simulink model "s_c856m4k"  (R2016b)
(part 2 of 92)

      settings: AttributesFormatString=Latency = %<latency>
      mask Display:
      | port_label('input', 1, 'd');
      | port_label('output', 1, 'q');
      | disp(['Z^-', num2str(latency)]);
  pipeline20 : Subsystem  AncestorBlock=casper_library_delays/pipeline  mask(pipeline){latency=2}
      mask help:
      | An explicitly laid-out delay line to avoid mapping to SRL16s
      | for use in pipelining to help achieve timing closure.
      mask init:
      | pipeline_init(gcb,'latency',latency);
      settings: AttributesFormatString=Latency = %<latency>
      mask Display:
      | port_label('input', 1, 'd');
      | port_label('output', 1, 'q');
      | disp(['Z^-', num2str(latency)]);
  pipeline21 : Subsystem  AncestorBlock=casper_library_delays/pipeline  mask(pipeline){latency=2}
      mask help:
      | An explicitly laid-out delay line to avoid mapping to SRL16s
      | for use in pipelining to help achieve timing closure.
      mask init:
      | pipeline_init(gcb,'latency',latency);
      settings: AttributesFormatString=Latency = %<latency>
      mask Display:
      | port_label('input', 1, 'd');
      | port_label('output', 1, 'q');
      | disp(['Z^-', num2str(latency)]);
  pipeline22 : Subsystem  AncestorBlock=casper_library_delays/pipeline  mask(pipeline){latency=2}
      mask help:
      | An explicitly laid-out delay line to avoid mapping to SRL16s
      | for use in pipelining to help achieve timing closure.
      mask init:
      | pipeline_init(gcb,'latency',latency);
      settings: AttributesFormatString=Latency = %<latency>
      mask Display:
      | port_label('input', 1, 'd');
      | port_label('output', 1, 'q');
      | disp(['Z^-', num2str(latency)]);
  pipeline23 : Subsystem  AncestorBlock=casper_library_delays/pipeline  mask(pipeline){latency=2}
      mask help:
      | An explicitly laid-out delay line to avoid mapping to SRL16s
      | for use in pipelining to help achieve timing closure.
      mask init:
      | pipeline_init(gcb,'latency',latency);
      settings: AttributesFormatString=Latency = %<latency>
      mask Display:
      | port_label('input', 1, 'd');
      | port_label('output', 1, 'q');
      | disp(['Z^-', num2str(latency)]);
  pipeline24 : Subsystem  AncestorBlock=casper_library_delays/pipeline  mask(pipeline){latency=2}
      mask help:
      | An explicitly laid-out delay line to avoid mapping to SRL16s
      | for use in pipelining to help achieve timing closure.
      mask init:
      | pipeline_init(gcb,'latency',latency);
      settings: AttributesFormatString=Latency = %<latency>
      mask Display:
      | port_label('input', 1, 'd');
      | port_label('output', 1, 'q');
      | disp(['Z^-', num2str(latency)]);
  pipeline25 : Subsystem  AncestorBlock=casper_library_delays/pipeline  mask(pipeline){latency=2}
      mask help:
      | An explicitly laid-out delay line to avoid mapping to SRL16s
      | for use in pipelining to help achieve timing closure.
      mask init:
      | pipeline_init(gcb,'latency',latency);
      settings: AttributesFormatString=Latency = %<latency>
      mask Display:
      | port_label('input', 1, 'd');
      | port_label('output', 1, 'q');
      | disp(['Z^-', num2str(latency)]);
  pipeline26 : Subsystem  AncestorBlock=casper_library_delays/pipeline  mask(pipeline){latency=2}
      mask help:
      | An explicitly laid-out delay line to avoid mapping to SRL16s
      | for use in pipelining to help achieve timing closure.
      mask init:
      | pipeline_init(gcb,'latency',latency);
      settings: AttributesFormatString=Latency = %<latency>
      mask Display:
      | port_label('input', 1, 'd');
      | port_label('output', 1, 'q');
      | disp(['Z^-', num2str(latency)]);
  pipeline27 : Subsystem  AncestorBlock=casper_library_delays/pipeline  mask(pipeline){latency=2}
      mask help:
      | An explicitly laid-out delay line to avoid mapping to SRL16s
      | for use in pipelining to help achieve timing closure.
      mask init:
      | pipeline_init(gcb,'latency',latency);
      settings: AttributesFormatString=Latency = %<latency>
      mask Display:
      | port_label('input', 1, 'd');
      | port_label('output', 1, 'q');
      | disp(['Z^-', num2str(latency)]);
  pipeline28 : Subsystem  AncestorBlock=casper_library_delays/pipeline  mask(pipeline){latency=2}
      mask help:
      | An explicitly laid-out delay line to avoid mapping to SRL16s
      | for use in pipelining to help achieve timing closure.
      mask init:
      | pipeline_init(gcb,'latency',latency);
      settings: AttributesFormatString=Latency = %<latency>
      mask Display:
      | port_label('input', 1, 'd');
      | port_label('output', 1, 'q');
      | disp(['Z^-', num2str(latency)]);
  pipeline29 : Subsystem  AncestorBlock=casper_library_delays/pipeline  mask(pipeline){latency=2}
      mask help:
      | An explicitly laid-out delay line to avoid mapping to SRL16s
      | for use in pipelining to help achieve timing closure.
      mask init:
      | pipeline_init(gcb,'latency',latency);
      settings: AttributesFormatString=Latency = %<latency>
      mask Display:
      | port_label('input', 1, 'd');
      | port_label('output', 1, 'q');
      | disp(['Z^-', num2str(latency)]);
  pipeline3 : Subsystem  AncestorBlock=casper_library_delays/pipeline  mask(pipeline){latency=2}
      mask help:
      | An explicitly laid-out delay line to avoid mapping to SRL16s
      | for use in pipelining to help achieve timing closure.
      mask init:
      | pipeline_init(gcb,'latency',latency);
      settings: AttributesFormatString=Latency = %<latency>
      mask Display:
      | port_label('input', 1, 'd');
      | port_label('output', 1, 'q');
      | disp(['Z^-', num2str(latency)]);
  pipeline30 : Subsystem  AncestorBlock=casper_library_delays/pipeline  mask(pipeline){latency=2}
      mask help:
      | An explicitly laid-out delay line to avoid mapping to SRL16s
      | for use in pipelining to help achieve timing closure.
      mask init:
      | pipeline_init(gcb,'latency',latency);
      settings: AttributesFormatString=Latency = %<latency>
      mask Display:
      | port_label('input', 1, 'd');
      | port_label('output', 1, 'q');
      | disp(['Z^-', num2str(latency)]);
  pipeline31 : Subsystem  AncestorBlock=casper_library_delays/pipeline  mask(pipeline){latency=2}
      mask help:
      | An explicitly laid-out delay line to avoid mapping to SRL16s
      | for use in pipelining to help achieve timing closure.
      mask init:
      | pipeline_init(gcb,'latency',latency);
      settings: AttributesFormatString=Latency = %<latency>
      mask Display:
      | port_label('input', 1, 'd');
      | port_label('output', 1, 'q');
      | disp(['Z^-', num2str(latency)]);
  pipeline32 : Subsystem  AncestorBlock=casper_library_delays/pipeline  mask(pipeline){latency=2}
      mask help:
      | An explicitly laid-out delay line to avoid mapping to SRL16s
      | for use in pipelining to help achieve timing closure.
      mask init:
      | pipeline_init(gcb,'latency',latency);
      settings: AttributesFormatString=Latency = %<latency>
      mask Display:
      | port_label('input', 1, 'd');
      | port_label('output', 1, 'q');
      | disp(['Z^-', num2str(latency)]);
  pipeline33 : Subsystem  AncestorBlock=casper_library_delays/pipeline  mask(pipeline){latency=2}
      mask help:
      | An explicitly laid-out delay line to avoid mapping to SRL16s
      | for use in pipelining to help achieve timing closure.
      mask init:
      | pipeline_init(gcb,'latency',latency);
      settings: AttributesFormatString=Latency = %<latency>
      mask Display:
      | port_label('input', 1, 'd');
      | port_label('output', 1, 'q');
      | disp(['Z^-', num2str(latency)]);
  pipeline34 : Subsystem  AncestorBlock=casper_library_delays/pipeline  mask(pipeline){latency=2}
      mask help:
      | An explicitly laid-out delay line to avoid mapping to SRL16s
      | for use in pipelining to help achieve timing closure.
      mask init:
      | pipeline_init(gcb,'latency',latency);
      settings: AttributesFormatString=Latency = %<latency>
      mask Display:
      | port_label('input', 1, 'd');
      | port_label('output', 1, 'q');
      | disp(['Z^-', num2str(latency)]);
  pipeline35 : Subsystem  AncestorBlock=casper_library_delays/pipeline  mask(pipeline){latency=2}
      mask help:
      | An explicitly laid-out delay line to avoid mapping to SRL16s
      | for use in pipelining to help achieve timing closure.
      mask init:
      | pipeline_init(gcb,'latency',latency);
      settings: AttributesFormatString=Latency = %<latency>
      mask Display:
      | port_label('input', 1, 'd');
      | port_label('output', 1, 'q');
      | disp(['Z^-', num2str(latency)]);
  pipeline36 : Subsystem  AncestorBlock=casper_library_delays/pipeline  mask(pipeline){latency=2}
      mask help:
      | An explicitly laid-out delay line to avoid mapping to SRL16s
      | for use in pipelining to help achieve timing closure.
      mask init:
      | pipeline_init(gcb,'latency',latency);
      settings: AttributesFormatString=Latency = %<latency>
      mask Display:
      | port_label('input', 1, 'd');
      | port_label('output', 1, 'q');
      | disp(['Z^-', num2str(latency)]);
  pipeline37 : Subsystem  AncestorBlock=casper_library_delays/pipeline  mask(pipeline){latency=2}
      mask help:
      | An explicitly laid-out delay line to avoid mapping to SRL16s
      | for use in pipelining to help achieve timing closure.
      mask init:
      | pipeline_init(gcb,'latency',latency);
      settings: AttributesFormatString=Latency = %<latency>
      mask Display:
      | port_label('input', 1, 'd');
      | port_label('output', 1, 'q');
      | disp(['Z^-', num2str(latency)]);
  pipeline38 : Subsystem  AncestorBlock=casper_library_delays/pipeline  mask(pipeline){latency=2}
      mask help:
      | An explicitly laid-out delay line to avoid mapping to SRL16s
      | for use in pipelining to help achieve timing closure.
      mask init:
      | pipeline_init(gcb,'latency',latency);
      settings: AttributesFormatString=Latency = %<latency>
      mask Display:
      | port_label('input', 1, 'd');
      | port_label('output', 1, 'q');
      | disp(['Z^-', num2str(latency)]);
  pipeline39 : Subsystem  AncestorBlock=casper_library_delays/pipeline  mask(pipeline){latency=2}
      mask help:
      | An explicitly laid-out delay line to avoid mapping to SRL16s
      | for use in pipelining to help achieve timing closure.
      mask init:
      | pipeline_init(gcb,'latency',latency);
      settings: AttributesFormatString=Latency = %<latency>
      mask Display:
      | port_label('input', 1, 'd');
      | port_label('output', 1, 'q');
      | disp(['Z^-', num2str(latency)]);
  pipeline4 : Subsystem  AncestorBlock=casper_library_delays/pipeline  mask(pipeline){latency=2}
      mask help:
      | An explicitly laid-out delay line to avoid mapping to SRL16s
      | for use in pipelining to help achieve timing closure.
      mask init:
      | pipeline_init(gcb,'latency',latency);
      settings: AttributesFormatString=Latency = %<latency>
      mask Display:
      | port_label('input', 1, 'd');
      | port_label('output', 1, 'q');
      | disp(['Z^-', num2str(latency)]);
  pipeline40 : Subsystem  AncestorBlock=casper_library_delays/pipeline  mask(pipeline){latency=2}
      mask help:
      | An explicitly laid-out delay line to avoid mapping to SRL16s
      | for use in pipelining to help achieve timing closure.
      mask init:
      | pipeline_init(gcb,'latency',latency);
      settings: AttributesFormatString=Latency = %<latency>
      mask Display:
      | port_label('input', 1, 'd');
      | port_label('output', 1, 'q');
      | disp(['Z^-', num2str(latency)]);
  pipeline41 : Subsystem  AncestorBlock=casper_library_delays/pipeline  mask(pipeline){latency=2}
      mask help:
      | An explicitly laid-out delay line to avoid mapping to SRL16s
      | for use in pipelining to help achieve timing closure.
      mask init:
      | pipeline_init(gcb,'latency',latency);
      settings: AttributesFormatString=Latency = %<latency>
      mask Display:
      | port_label('input', 1, 'd');
      | port_label('output', 1, 'q');
      | disp(['Z^-', num2str(latency)]);
  pipeline42 : Subsystem  AncestorBlock=casper_library_delays/pipeline  mask(pipeline){latency=2}
      mask help:
      | An explicitly laid-out delay line to avoid mapping to SRL16s
      | for use in pipelining to help achieve timing closure.
      mask init:
      | pipeline_init(gcb,'latency',latency);
      settings: AttributesFormatString=Latency = %<latency>
      mask Display:
      | port_label('input', 1, 'd');
      | port_label('output', 1, 'q');
      | disp(['Z^-', num2str(latency)]);
  pipeline43 : Subsystem  AncestorBlock=casper_library_delays/pipeline  mask(pipeline){latency=2}
      mask help:
      | An explicitly laid-out delay line to avoid mapping to SRL16s
      | for use in pipelining to help achieve timing closure.
      mask init:
      | pipeline_init(gcb,'latency',latency);
      settings: AttributesFormatString=Latency = %<latency>
      mask Display:
      | port_label('input', 1, 'd');
      | port_label('output', 1, 'q');
      | disp(['Z^-', num2str(latency)]);
  pipeline44 : Subsystem  AncestorBlock=casper_library_delays/pipeline  mask(pipeline){latency=2}
      mask help:
      | An explicitly laid-out delay line to avoid mapping to SRL16s
      | for use in pipelining to help achieve timing closure.
      mask init:
      | pipeline_init(gcb,'latency',latency);
      settings: AttributesFormatString=Latency = %<latency>
      mask Display:
      | port_label('input', 1, 'd');
      | port_label('output', 1, 'q');
      | disp(['Z^-', num2str(latency)]);
  pipeline45 : Subsystem  AncestorBlock=casper_library_delays/pipeline  mask(pipeline){latency=2}
      mask help:
      | An explicitly laid-out delay line to avoid mapping to SRL16s
      | for use in pipelining to help achieve timing closure.
      mask init:
      | pipeline_init(gcb,'latency',latency);
      settings: AttributesFormatString=Latency = %<latency>
      mask Display:
      | port_label('input', 1, 'd');
      | port_label('output', 1, 'q');
      | disp(['Z^-', num2str(latency)]);
  pipeline46 : Subsystem  AncestorBlock=casper_library_delays/pipeline  mask(pipeline){latency=2}
      mask help:
      | An explicitly laid-out delay line to avoid mapping to SRL16s
      | for use in pipelining to help achieve timing closure.
      mask init:
      | pipeline_init(gcb,'latency',latency);
      settings: AttributesFormatString=Latency = %<latency>
      mask Display:
      | port_label('input', 1, 'd');
      | port_label('output', 1, 'q');
      | disp(['Z^-', num2str(latency)]);
  pipeline47 : Subsystem  AncestorBlock=casper_library_delays/pipeline  mask(pipeline){latency=2}
      mask help:
      | An explicitly laid-out delay line to avoid mapping to SRL16s
      | for use in pipelining to help achieve timing closure.
      mask init:
      | pipeline_init(gcb,'latency',latency);
      settings: AttributesFormatString=Latency = %<latency>
      mask Display:
      | port_label('input', 1, 'd');
      | port_label('output', 1, 'q');
      | disp(['Z^-', num2str(latency)]);
  pipeline48 : Subsystem  AncestorBlock=casper_library_delays/pipeline  mask(pipeline){latency=2}
      mask help:
      | An explicitly laid-out delay line to avoid mapping to SRL16s
      | for use in pipelining to help achieve timing closure.
      mask init:
      | pipeline_init(gcb,'latency',latency);
      settings: AttributesFormatString=Latency = %<latency>
      mask Display:
      | port_label('input', 1, 'd');
      | port_label('output', 1, 'q');
      | disp(['Z^-', num2str(latency)]);
  pipeline49 : Subsystem  AncestorBlock=casper_library_delays/pipeline  mask(pipeline){latency=2}
      mask help:
      | An explicitly laid-out delay line to avoid mapping to SRL16s
      | for use in pipelining to help achieve timing closure.
      mask init:
      | pipeline_init(gcb,'latency',latency);
      settings: AttributesFormatString=Latency = %<latency>
      mask Display:
      | port_label('input', 1, 'd');
      | port_label('output', 1, 'q');
      | disp(['Z^-', num2str(latency)]);
  pipeline5 : Subsystem  AncestorBlock=casper_library_delays/pipeline  mask(pipeline){latency=2}
      mask help:
      | An explicitly laid-out delay line to avoid mapping to SRL16s
      | for use in pipelining to help achieve timing closure.
      mask init:
      | pipeline_init(gcb,'latency',latency);
      settings: AttributesFormatString=Latency = %<latency>
      mask Display:
      | port_label('input', 1, 'd');
      | port_label('output', 1, 'q');
      | disp(['Z^-', num2str(latency)]);
  pipeline50 : Subsystem  AncestorBlock=casper_library_delays/pipeline  mask(pipeline){latency=2}
      mask help:
      | An explicitly laid-out delay line to avoid mapping to SRL16s
      | for use in pipelining to help achieve timing closure.
      mask init:
      | pipeline_init(gcb,'latency',latency);
      settings: AttributesFormatString=Latency = %<latency>
      mask Display:
      | port_label('input', 1, 'd');
      | port_label('output', 1, 'q');
      | disp(['Z^-', num2str(latency)]);
  pipeline51 : Subsystem  AncestorBlock=casper_library_delays/pipeline  mask(pipeline){latency=2}
      mask help:
      | An explicitly laid-out delay line to avoid mapping to SRL16s
      | for use in pipelining to help achieve timing closure.
      mask init:
      | pipeline_init(gcb,'latency',latency);
      settings: AttributesFormatString=Latency = %<latency>
      mask Display:
      | port_label('input', 1, 'd');
      | port_label('output', 1, 'q');
      | disp(['Z^-', num2str(latency)]);
  pipeline52 : Subsystem  AncestorBlock=casper_library_delays/pipeline  mask(pipeline){latency=2}
      mask help:
      | An explicitly laid-out delay line to avoid mapping to SRL16s
      | for use in pipelining to help achieve timing closure.
      mask init:
      | pipeline_init(gcb,'latency',latency);
      settings: AttributesFormatString=Latency = %<latency>
      mask Display:
      | port_label('input', 1, 'd');
      | port_label('output', 1, 'q');
      | disp(['Z^-', num2str(latency)]);
  pipeline53 : Subsystem  AncestorBlock=casper_library_delays/pipeline  mask(pipeline){latency=2}
      mask help:
      | An explicitly laid-out delay line to avoid mapping to SRL16s
      | for use in pipelining to help achieve timing closure.
      mask init:
      | pipeline_init(gcb,'latency',latency);
      settings: AttributesFormatString=Latency = %<latency>
      mask Display:
      | port_label('input', 1, 'd');
      | port_label('output', 1, 'q');
      | disp(['Z^-', num2str(latency)]);
  pipeline54 : Subsystem  AncestorBlock=casper_library_delays/pipeline  mask(pipeline){latency=2}
      mask help:
      | An explicitly laid-out delay line to avoid mapping to SRL16s
      | for use in pipelining to help achieve timing closure.
      mask init:
      | pipeline_init(gcb,'latency',latency);
      settings: AttributesFormatString=Latency = %<latency>
      mask Display:
      | port_label('input', 1, 'd');
      | port_label('output', 1, 'q');
      | disp(['Z^-', num2str(latency)]);
  pipeline55 : Subsystem  AncestorBlock=casper_library_delays/pipeline  mask(pipeline){latency=2}
      mask help:
      | An explicitly laid-out delay line to avoid mapping to SRL16s
      | for use in pipelining to help achieve timing closure.
      mask init:
      | pipeline_init(gcb,'latency',latency);
      settings: AttributesFormatString=Latency = %<latency>
      mask Display:
      | port_label('input', 1, 'd');
      | port_label('output', 1, 'q');
      | disp(['Z^-', num2str(latency)]);
  pipeline56 : Subsystem  AncestorBlock=casper_library_delays/pipeline  mask(pipeline){latency=2}
      mask help:
      | An explicitly laid-out delay line to avoid mapping to SRL16s
      | for use in pipelining to help achieve timing closure.
      mask init:
      | pipeline_init(gcb,'latency',latency);
      settings: AttributesFormatString=Latency = %<latency>
      mask Display:
      | port_label('input', 1, 'd');
      | port_label('output', 1, 'q');
      | disp(['Z^-', num2str(latency)]);
  pipeline57 : Subsystem  AncestorBlock=casper_library_delays/pipeline  mask(pipeline){latency=2}
      mask help:
      | An explicitly laid-out delay line to avoid mapping to SRL16s
      | for use in pipelining to help achieve timing closure.
      mask init:
      | pipeline_init(gcb,'latency',latency);
      settings: AttributesFormatString=Latency = %<latency>
      mask Display:
      | port_label('input', 1, 'd');
      | port_label('output', 1, 'q');
      | disp(['Z^-', num2str(latency)]);
  pipeline58 : Subsystem  AncestorBlock=casper_library_delays/pipeline  mask(pipeline){latency=2}
      mask help:
      | An explicitly laid-out delay line to avoid mapping to SRL16s
      | for use in pipelining to help achieve timing closure.
      mask init:
      | pipeline_init(gcb,'latency',latency);
      settings: AttributesFormatString=Latency = %<latency>
      mask Display:
      | port_label('input', 1, 'd');
      | port_label('output', 1, 'q');
      | disp(['Z^-', num2str(latency)]);
  pipeline59 : Subsystem  AncestorBlock=casper_library_delays/pipeline  mask(pipeline){latency=2}
      mask help:
      | An explicitly laid-out delay line to avoid mapping to SRL16s
      | for use in pipelining to help achieve timing closure.
      mask init:
      | pipeline_init(gcb,'latency',latency);
      settings: AttributesFormatString=Latency = %<latency>
      mask Display:
      | port_label('input', 1, 'd');
      | port_label('output', 1, 'q');
      | disp(['Z^-', num2str(latency)]);
  pipeline6 : Subsystem  AncestorBlock=casper_library_delays/pipeline  mask(pipeline){latency=2}
      mask help:
      | An explicitly laid-out delay line to avoid mapping to SRL16s
      | for use in pipelining to help achieve timing closure.
      mask init:
      | pipeline_init(gcb,'latency',latency);
      settings: AttributesFormatString=Latency = %<latency>
      mask Display:
      | port_label('input', 1, 'd');
      | port_label('output', 1, 'q');
      | disp(['Z^-', num2str(latency)]);
  pipeline60 : Subsystem  AncestorBlock=casper_library_delays/pipeline  mask(pipeline){latency=2}
      mask help:
      | An explicitly laid-out delay line to avoid mapping to SRL16s
      | for use in pipelining to help achieve timing closure.
      mask init:
      | pipeline_init(gcb,'latency',latency);
      settings: AttributesFormatString=Latency = %<latency>
      mask Display:
      | port_label('input', 1, 'd');
      | port_label('output', 1, 'q');
      | disp(['Z^-', num2str(latency)]);
  pipeline61 : Subsystem  AncestorBlock=casper_library_delays/pipeline  mask(pipeline){latency=2}
      mask help:
      | An explicitly laid-out delay line to avoid mapping to SRL16s
      | for use in pipelining to help achieve timing closure.
      mask init:
      | pipeline_init(gcb,'latency',latency);
      settings: AttributesFormatString=Latency = %<latency>
      mask Display:
      | port_label('input', 1, 'd');
      | port_label('output', 1, 'q');
      | disp(['Z^-', num2str(latency)]);
  pipeline62 : Subsystem  AncestorBlock=casper_library_delays/pipeline  mask(pipeline){latency=2}
      mask help:
      | An explicitly laid-out delay line to avoid mapping to SRL16s
      | for use in pipelining to help achieve timing closure.
      mask init:
      | pipeline_init(gcb,'latency',latency);
      settings: AttributesFormatString=Latency = %<latency>
      mask Display:
      | port_label('input', 1, 'd');
      | port_label('output', 1, 'q');
      | disp(['Z^-', num2str(latency)]);
  pipeline63 : Subsystem  AncestorBlock=casper_library_delays/pipeline  mask(pipeline){latency=2}
      mask help:
      | An explicitly laid-out delay line to avoid mapping to SRL16s
      | for use in pipelining to help achieve timing closure.
      mask init:
      | pipeline_init(gcb,'latency',latency);
      settings: AttributesFormatString=Latency = %<latency>
      mask Display:
      | port_label('input', 1, 'd');
      | port_label('output', 1, 'q');
      | disp(['Z^-', num2str(latency)]);
  pipeline64 : Subsystem  AncestorBlock=casper_library_delays/pipeline  mask(pipeline){latency=2}
      mask help:
      | An explicitly laid-out delay line to avoid mapping to SRL16s
      | for use in pipelining to help achieve timing closure.
      mask init:
      | pipeline_init(gcb,'latency',latency);
      settings: AttributesFormatString=Latency = %<latency>
      mask Display:
      | port_label('input', 1, 'd');
      | port_label('output', 1, 'q');
      | disp(['Z^-', num2str(latency)]);
  pipeline65 : Subsystem  AncestorBlock=casper_library_delays/pipeline  mask(pipeline){latency=1}
      mask help:
      | An explicitly laid-out delay line to avoid mapping to SRL16s
      | for use in pipelining to help achieve timing closure.
      mask init:
      | pipeline_init(gcb,'latency',latency);
      settings: AttributesFormatString=Latency = %<latency>
      mask Display:
      | port_label('input', 1, 'd');
      | port_label('output', 1, 'q');
      | disp(['Z^-', num2str(latency)]);
  pipeline66 : Subsystem  AncestorBlock=casper_library_delays/pipeline  mask(pipeline){latency=2}
      mask help:
      | An explicitly laid-out delay line to avoid mapping to SRL16s
      | for use in pipelining to help achieve timing closure.
      mask init:
      | pipeline_init(gcb,'latency',latency);
      settings: AttributesFormatString=Latency = %<latency>
      mask Display:
      | port_label('input', 1, 'd');
      | port_label('output', 1, 'q');
      | disp(['Z^-', num2str(latency)]);
  pipeline67 : Subsystem  AncestorBlock=casper_library_delays/pipeline  mask(pipeline){latency=2}
      mask help:
      | An explicitly laid-out delay line to avoid mapping to SRL16s
      | for use in pipelining to help achieve timing closure.
      mask init:
      | pipeline_init(gcb,'latency',latency);
      settings: AttributesFormatString=Latency = %<latency>
      mask Display:
      | port_label('input', 1, 'd');
      | port_label('output', 1, 'q');
      | disp(['Z^-', num2str(latency)]);
  pipeline68 : Subsystem  AncestorBlock=casper_library_delays/pipeline  mask(pipeline){latency=2}
      mask help:
      | An explicitly laid-out delay line to avoid mapping to SRL16s
      | for use in pipelining to help achieve timing closure.
      mask init:
      | pipeline_init(gcb,'latency',latency);
      settings: AttributesFormatString=Latency = %<latency>
      mask Display:
      | port_label('input', 1, 'd');
      | port_label('output', 1, 'q');
      | disp(['Z^-', num2str(latency)]);
  pipeline69 : Subsystem  AncestorBlock=casper_library_delays/pipeline  mask(pipeline){latency=2}
      mask help:
      | An explicitly laid-out delay line to avoid mapping to SRL16s
      | for use in pipelining to help achieve timing closure.
      mask init:
      | pipeline_init(gcb,'latency',latency);
      settings: AttributesFormatString=Latency = %<latency>
      mask Display:
      | port_label('input', 1, 'd');
      | port_label('output', 1, 'q');
      | disp(['Z^-', num2str(latency)]);
  pipeline7 : Subsystem  AncestorBlock=casper_library_delays/pipeline  mask(pipeline){latency=2}
      mask help:
      | An explicitly laid-out delay line to avoid mapping to SRL16s
      | for use in pipelining to help achieve timing closure.
      mask init:
      | pipeline_init(gcb,'latency',latency);
      settings: AttributesFormatString=Latency = %<latency>
      mask Display:
      | port_label('input', 1, 'd');
      | port_label('output', 1, 'q');
      | disp(['Z^-', num2str(latency)]);
  pipeline70 : Subsystem  AncestorBlock=casper_library_delays/pipeline  mask(pipeline){latency=2}
      mask help:
      | An explicitly laid-out delay line to avoid mapping to SRL16s
      | for use in pipelining to help achieve timing closure.
      mask init:
      | pipeline_init(gcb,'latency',latency);
      settings: AttributesFormatString=Latency = %<latency>
      mask Display:
      | port_label('input', 1, 'd');
      | port_label('output', 1, 'q');
      | disp(['Z^-', num2str(latency)]);
  pipeline71 : Subsystem  AncestorBlock=casper_library_delays/pipeline  mask(pipeline){latency=2}
      mask help:
      | An explicitly laid-out delay line to avoid mapping to SRL16s
      | for use in pipelining to help achieve timing closure.
      mask init:
      | pipeline_init(gcb,'latency',latency);
      settings: AttributesFormatString=Latency = %<latency>
      mask Display:
      | port_label('input', 1, 'd');
      | port_label('output', 1, 'q');
      | disp(['Z^-', num2str(latency)]);
  pipeline72 : Subsystem  AncestorBlock=casper_library_delays/pipeline  mask(pipeline){latency=2}
      mask help:
      | An explicitly laid-out delay line to avoid mapping to SRL16s
      | for use in pipelining to help achieve timing closure.
      mask init:
      | pipeline_init(gcb,'latency',latency);
      settings: AttributesFormatString=Latency = %<latency>
      mask Display:
      | port_label('input', 1, 'd');
      | port_label('output', 1, 'q');
      | disp(['Z^-', num2str(latency)]);
  pipeline73 : Subsystem  AncestorBlock=casper_library_delays/pipeline  mask(pipeline){latency=2}
      mask help:
      | An explicitly laid-out delay line to avoid mapping to SRL16s
      | for use in pipelining to help achieve timing closure.
      mask init:
      | pipeline_init(gcb,'latency',latency);
      settings: AttributesFormatString=Latency = %<latency>
      mask Display:
      | port_label('input', 1, 'd');
      | port_label('output', 1, 'q');
      | disp(['Z^-', num2str(latency)]);
  pipeline74 : Subsystem  AncestorBlock=casper_library_delays/pipeline  mask(pipeline){latency=2}
      mask help:
      | An explicitly laid-out delay line to avoid mapping to SRL16s
      | for use in pipelining to help achieve timing closure.
      mask init:
      | pipeline_init(gcb,'latency',latency);
      settings: AttributesFormatString=Latency = %<latency>
      mask Display:
      | port_label('input', 1, 'd');
      | port_label('output', 1, 'q');
      | disp(['Z^-', num2str(latency)]);
  pipeline75 : Subsystem  AncestorBlock=casper_library_delays/pipeline  mask(pipeline){latency=2}
      mask help:
      | An explicitly laid-out delay line to avoid mapping to SRL16s
      | for use in pipelining to help achieve timing closure.
      mask init:
      | pipeline_init(gcb,'latency',latency);
      settings: AttributesFormatString=Latency = %<latency>
      mask Display:
      | port_label('input', 1, 'd');
      | port_label('output', 1, 'q');
      | disp(['Z^-', num2str(latency)]);
  pipeline76 : Subsystem  AncestorBlock=casper_library_delays/pipeline  mask(pipeline){latency=2}
      mask help:
      | An explicitly laid-out delay line to avoid mapping to SRL16s
      | for use in pipelining to help achieve timing closure.
      mask init:
      | pipeline_init(gcb,'latency',latency);
      settings: AttributesFormatString=Latency = %<latency>
      mask Display:
      | port_label('input', 1, 'd');
      | port_label('output', 1, 'q');
      | disp(['Z^-', num2str(latency)]);
  pipeline77 : Subsystem  AncestorBlock=casper_library_delays/pipeline  mask(pipeline){latency=2}
      mask help:
      | An explicitly laid-out delay line to avoid mapping to SRL16s
      | for use in pipelining to help achieve timing closure.
      mask init:
      | pipeline_init(gcb,'latency',latency);
      settings: AttributesFormatString=Latency = %<latency>
      mask Display:
      | port_label('input', 1, 'd');
      | port_label('output', 1, 'q');
      | disp(['Z^-', num2str(latency)]);
  pipeline78 : Subsystem  AncestorBlock=casper_library_delays/pipeline  mask(pipeline){latency=2}
      mask help:
      | An explicitly laid-out delay line to avoid mapping to SRL16s
      | for use in pipelining to help achieve timing closure.
      mask init:
      | pipeline_init(gcb,'latency',latency);
      settings: AttributesFormatString=Latency = %<latency>
      mask Display:
      | port_label('input', 1, 'd');
      | port_label('output', 1, 'q');
      | disp(['Z^-', num2str(latency)]);
  pipeline79 : Subsystem  AncestorBlock=casper_library_delays/pipeline  mask(pipeline){latency=2}
      mask help:
      | An explicitly laid-out delay line to avoid mapping to SRL16s
      | for use in pipelining to help achieve timing closure.
      mask init:
      | pipeline_init(gcb,'latency',latency);
      settings: AttributesFormatString=Latency = %<latency>
      mask Display:
      | port_label('input', 1, 'd');
      | port_label('output', 1, 'q');
      | disp(['Z^-', num2str(latency)]);
  pipeline8 : Subsystem  AncestorBlock=casper_library_delays/pipeline  mask(pipeline){latency=2}
      mask help:
      | An explicitly laid-out delay line to avoid mapping to SRL16s
      | for use in pipelining to help achieve timing closure.
      mask init:
      | pipeline_init(gcb,'latency',latency);
      settings: AttributesFormatString=Latency = %<latency>
      mask Display:
      | port_label('input', 1, 'd');
      | port_label('output', 1, 'q');
      | disp(['Z^-', num2str(latency)]);
  pipeline80 : Subsystem  AncestorBlock=casper_library_delays/pipeline  mask(pipeline){latency=2}
      mask help:
      | An explicitly laid-out delay line to avoid mapping to SRL16s
      | for use in pipelining to help achieve timing closure.
      mask init:
      | pipeline_init(gcb,'latency',latency);
      settings: AttributesFormatString=Latency = %<latency>
      mask Display:
      | port_label('input', 1, 'd');
      | port_label('output', 1, 'q');
      | disp(['Z^-', num2str(latency)]);
  pipeline81 : Subsystem  AncestorBlock=casper_library_delays/pipeline  mask(pipeline){latency=2}
      mask help:
      | An explicitly laid-out delay line to avoid mapping to SRL16s
      | for use in pipelining to help achieve timing closure.
      mask init:
      | pipeline_init(gcb,'latency',latency);
      settings: AttributesFormatString=Latency = %<latency>
      mask Display:
      | port_label('input', 1, 'd');
      | port_label('output', 1, 'q');
      | disp(['Z^-', num2str(latency)]);
  pipeline82 : Subsystem  AncestorBlock=casper_library_delays/pipeline  mask(pipeline){latency=2}
      mask help:
      | An explicitly laid-out delay line to avoid mapping to SRL16s
      | for use in pipelining to help achieve timing closure.
      mask init:
      | pipeline_init(gcb,'latency',latency);
      settings: AttributesFormatString=Latency = %<latency>
      mask Display:
      | port_label('input', 1, 'd');
      | port_label('output', 1, 'q');
      | disp(['Z^-', num2str(latency)]);
  pipeline83 : Subsystem  AncestorBlock=casper_library_delays/pipeline  mask(pipeline){latency=2}
      mask help:
      | An explicitly laid-out delay line to avoid mapping to SRL16s
      | for use in pipelining to help achieve timing closure.
      mask init:
      | pipeline_init(gcb,'latency',latency);
      settings: AttributesFormatString=Latency = %<latency>
      mask Display:
      | port_label('input', 1, 'd');
      | port_label('output', 1, 'q');
      | disp(['Z^-', num2str(latency)]);
  pipeline84 : Subsystem  AncestorBlock=casper_library_delays/pipeline  mask(pipeline){latency=2}
      mask help:
      | An explicitly laid-out delay line to avoid mapping to SRL16s
      | for use in pipelining to help achieve timing closure.
      mask init:
      | pipeline_init(gcb,'latency',latency);
      settings: AttributesFormatString=Latency = %<latency>
      mask Display:
      | port_label('input', 1, 'd');
      | port_label('output', 1, 'q');
      | disp(['Z^-', num2str(latency)]);
  pipeline85 : Subsystem  AncestorBlock=casper_library_delays/pipeline  mask(pipeline){latency=2}
      mask help:
      | An explicitly laid-out delay line to avoid mapping to SRL16s
      | for use in pipelining to help achieve timing closure.
      mask init:
      | pipeline_init(gcb,'latency',latency);
      settings: AttributesFormatString=Latency = %<latency>
      mask Display:
      | port_label('input', 1, 'd');
      | port_label('output', 1, 'q');
      | disp(['Z^-', num2str(latency)]);
  pipeline86 : Subsystem  AncestorBlock=casper_library_delays/pipeline  mask(pipeline){latency=2}
      mask help:
      | An explicitly laid-out delay line to avoid mapping to SRL16s
      | for use in pipelining to help achieve timing closure.
      mask init:
      | pipeline_init(gcb,'latency',latency);
      settings: AttributesFormatString=Latency = %<latency>
      mask Display:
      | port_label('input', 1, 'd');
      | port_label('output', 1, 'q');
      | disp(['Z^-', num2str(latency)]);
  pipeline87 : Subsystem  AncestorBlock=casper_library_delays/pipeline  mask(pipeline){latency=2}
      mask help:
      | An explicitly laid-out delay line to avoid mapping to SRL16s
      | for use in pipelining to help achieve timing closure.
      mask init:
      | pipeline_init(gcb,'latency',latency);
      settings: AttributesFormatString=Latency = %<latency>
      mask Display:
      | port_label('input', 1, 'd');
      | port_label('output', 1, 'q');
      | disp(['Z^-', num2str(latency)]);
  pipeline88 : Subsystem  AncestorBlock=casper_library_delays/pipeline  mask(pipeline){latency=2}
      mask help:
      | An explicitly laid-out delay line to avoid mapping to SRL16s
      | for use in pipelining to help achieve timing closure.
      mask init:
      | pipeline_init(gcb,'latency',latency);
      settings: AttributesFormatString=Latency = %<latency>
      mask Display:
      | port_label('input', 1, 'd');
      | port_label('output', 1, 'q');
      | disp(['Z^-', num2str(latency)]);
  pipeline89 : Subsystem  AncestorBlock=casper_library_delays/pipeline  mask(pipeline){latency=2}
      mask help:
      | An explicitly laid-out delay line to avoid mapping to SRL16s
      | for use in pipelining to help achieve timing closure.
      mask init:
      | pipeline_init(gcb,'latency',latency);
      settings: AttributesFormatString=Latency = %<latency>
      mask Display:
      | port_label('input', 1, 'd');
      | port_label('output', 1, 'q');
      | disp(['Z^-', num2str(latency)]);
  pipeline9 : Subsystem  AncestorBlock=casper_library_delays/pipeline  mask(pipeline){latency=2}
      mask help:
      | An explicitly laid-out delay line to avoid mapping to SRL16s
      | for use in pipelining to help achieve timing closure.
      mask init:
      | pipeline_init(gcb,'latency',latency);
      settings: AttributesFormatString=Latency = %<latency>
      mask Display:
      | port_label('input', 1, 'd');
      | port_label('output', 1, 'q');
      | disp(['Z^-', num2str(latency)]);
  pipeline90 : Subsystem  AncestorBlock=casper_library_delays/pipeline  mask(pipeline){latency=2}
      mask help:
      | An explicitly laid-out delay line to avoid mapping to SRL16s
      | for use in pipelining to help achieve timing closure.
      mask init:
      | pipeline_init(gcb,'latency',latency);
      settings: AttributesFormatString=Latency = %<latency>
      mask Display:
      | port_label('input', 1, 'd');
      | port_label('output', 1, 'q');
      | disp(['Z^-', num2str(latency)]);
  pipeline91 : Subsystem  AncestorBlock=casper_library_delays/pipeline  mask(pipeline){latency=2}
      mask help:
      | An explicitly laid-out delay line to avoid mapping to SRL16s
      | for use in pipelining to help achieve timing closure.
      mask init:
      | pipeline_init(gcb,'latency',latency);
      settings: AttributesFormatString=Latency = %<latency>
      mask Display:
      | port_label('input', 1, 'd');
      | port_label('output', 1, 'q');
      | disp(['Z^-', num2str(latency)]);
  pipeline92 : Subsystem  AncestorBlock=casper_library_delays/pipeline  mask(pipeline){latency=2}
      mask help:
      | An explicitly laid-out delay line to avoid mapping to SRL16s
      | for use in pipelining to help achieve timing closure.
      mask init:
      | pipeline_init(gcb,'latency',latency);
      settings: AttributesFormatString=Latency = %<latency>
      mask Display:
      | port_label('input', 1, 'd');
      | port_label('output', 1, 'q');
      | disp(['Z^-', num2str(latency)]);
  pipeline93 : Subsystem  AncestorBlock=casper_library_delays/pipeline  mask(pipeline){latency=2}
      mask help:
      | An explicitly laid-out delay line to avoid mapping to SRL16s
      | for use in pipelining to help achieve timing closure.
      mask init:
      | pipeline_init(gcb,'latency',latency);
      settings: AttributesFormatString=Latency = %<latency>
      mask Display:
      | port_label('input', 1, 'd');
      | port_label('output', 1, 'q');
      | disp(['Z^-', num2str(latency)]);
  pipeline94 : Subsystem  AncestorBlock=casper_library_delays/pipeline  mask(pipeline){latency=2}
      mask help:
      | An explicitly laid-out delay line to avoid mapping to SRL16s
      | for use in pipelining to help achieve timing closure.
      mask init:
      | pipeline_init(gcb,'latency',latency);
      settings: AttributesFormatString=Latency = %<latency>
      mask Display:
      | port_label('input', 1, 'd');
      | port_label('output', 1, 'q');
      | disp(['Z^-', num2str(latency)]);
  pipeline95 : Subsystem  AncestorBlock=casper_library_delays/pipeline  mask(pipeline){latency=2}
      mask help:
      | An explicitly laid-out delay line to avoid mapping to SRL16s
      | for use in pipelining to help achieve timing closure.
      mask init:
      | pipeline_init(gcb,'latency',latency);
      settings: AttributesFormatString=Latency = %<latency>
      mask Display:
      | port_label('input', 1, 'd');
      | port_label('output', 1, 'q');
      | disp(['Z^-', num2str(latency)]);
  pipeline96 : Subsystem  AncestorBlock=casper_library_delays/pipeline  mask(pipeline){latency=2}
      mask help:
      | An explicitly laid-out delay line to avoid mapping to SRL16s
      | for use in pipelining to help achieve timing closure.
      mask init:
      | pipeline_init(gcb,'latency',latency);
      settings: AttributesFormatString=Latency = %<latency>
      mask Display:
      | port_label('input', 1, 'd');
      | port_label('output', 1, 'q');
      | disp(['Z^-', num2str(latency)]);
  pipeline97 : Subsystem  AncestorBlock=casper_library_delays/pipeline  mask(pipeline){latency=2}
      mask help:
      | An explicitly laid-out delay line to avoid mapping to SRL16s
      | for use in pipelining to help achieve timing closure.
      mask init:
      | pipeline_init(gcb,'latency',latency);
      settings: AttributesFormatString=Latency = %<latency>
      mask Display:
      | port_label('input', 1, 'd');
      | port_label('output', 1, 'q');
      | disp(['Z^-', num2str(latency)]);
  pipeline98 : Subsystem  AncestorBlock=casper_library_delays/pipeline  mask(pipeline){latency=2}
      mask help:
      | An explicitly laid-out delay line to avoid mapping to SRL16s
      | for use in pipelining to help achieve timing closure.
      mask init:
      | pipeline_init(gcb,'latency',latency);
      settings: AttributesFormatString=Latency = %<latency>
      mask Display:
      | port_label('input', 1, 'd');
      | port_label('output', 1, 'q');
      | disp(['Z^-', num2str(latency)]);
  pipeline99 : Subsystem  AncestorBlock=casper_library_delays/pipeline  mask(pipeline){latency=2}
      mask help:
      | An explicitly laid-out delay line to avoid mapping to SRL16s
      | for use in pipelining to help achieve timing closure.
      mask init:
      | pipeline_init(gcb,'latency',latency);
      settings: AttributesFormatString=Latency = %<latency>
      mask Display:
      | port_label('input', 1, 'd');
      | port_label('output', 1, 'q');
      | disp(['Z^-', num2str(latency)]);
  pktlen_check : Subsystem  mask{block_len=32}
      mask prompts: block_len "Expected length"
      mask Display:
      | disp(sprintf('block_len == %i?', block_len));
      | color('green');
      | port_label('input', 1, 'pktstart')
      | port_label('input', 2, 'dv')
      | color('red');
      | port_label('output', 1, 'err')
  qt_block_check : Subsystem  mask{block_len=512}
      mask prompts: block_len "Expected length"
      mask Display:
      | disp(sprintf('block_len == %i?', block_len));
      | color('green');
      | port_label('input', 1, 'dv')
      | color('red');
      | port_label('output', 1, 'err')
  qt_dv_err : Subsystem  Tag=xps:sw_reg  AncestorBlock=xps_library/software_register  mask(swreg){io_dir=To Processor, io_delay=0, sample_period=1, names=[dvblock_err_cnt], bitwidths=16, bin_pts=0, arith_types=0, sim_port=off, show_format=on}
      mask prompts: io_dir "I/O direction"; io_delay "I/O delay"; sample_period "Sample period"; names "Bitfield names [msb...lsb]"; bitwidths "Bitfield widths"; bin_pts "Bitfield binary pts"; arith_types "Bitfield types, ufix=0, fix=1, bool=2"; sim_port "Provide sim input/output?"; show_format "Print format string?"
      mask help: A 32-bit software-accessible register. Can be divided into bitfields of varying widths and types using the fields in the block mask.
      mask init:
      | swreg_init(gcb)
      settings: AttributesFormatString=1output:uf16.0 = 16 bits
      mask TypeOptions io_dir: To Processor | From Processor
      mask Callback io_dir:
      | mask_enables = get_param(gcb, 'MaskEnables');
      | mask_names = get_param(gcb, 'MaskNames');
      | if strcmp(get_param(gcb, 'io_dir'), 'To Processor'),
      |     mask_enables{ismember(mask_names, 'sample_period')} = 'off';
      | else
      |     mask_enables{ismember(mask_names, 'sample_period')} = 'on';
      | end
      | set_param(gcb, 'MaskEnables', mask_enables);
  quant0 : Subsystem  mask{channel_bits=fft_stages-1, din_bit_width=18, din_bin_pt=17, coeff_bit_width=16, coeff_bin_pt=1, dout_bit_width=8, dout_bin_pt=7, overflow=Saturate, quantization=Round  (unbiased: even values), conv_latency=4, add_latency=2, mult_latency=3, bram_latency=2}
      mask prompts: channel_bits "Number channels (2^?)"; din_bit_width "Data input bit width"; din_bin_pt "Data input binary point"; coeff_bit_width "Coefficient bit width"; coeff_bin_pt "Coefficient binary point"; dout_bit_width "Data out bit width"; dout_bin_pt "Data out binary point"; overflow "Overflow behaviour"; quantization "Quantization Behaviour"; conv_latency "Conversion latency"; add_latency "Adder latency"; mult_latency "Multiplier latency"; bram_latency "BRAM latency"
      mask TypeOptions overflow: Wrap | Saturate | Error
      mask TypeOptions quantization: Truncate | Round  (unbiased: +/- Inf) | Round  (unbiased: even values)
  quant1 : Subsystem  mask{channel_bits=fft_stages-1, din_bit_width=18, din_bin_pt=17, coeff_bit_width=16, coeff_bin_pt=1, dout_bit_width=8, dout_bin_pt=7, overflow=Saturate, quantization=Round  (unbiased: even values), conv_latency=4, add_latency=2, mult_latency=3, bram_latency=2}
      mask prompts: channel_bits "Number channels (2^?)"; din_bit_width "Data input bit width"; din_bin_pt "Data input binary point"; coeff_bit_width "Coefficient bit width"; coeff_bin_pt "Coefficient binary point"; dout_bit_width "Data out bit width"; dout_bin_pt "Data out binary point"; overflow "Overflow behaviour"; quantization "Quantization Behaviour"; conv_latency "Conversion latency"; add_latency "Adder latency"; mult_latency "Multiplier latency"; bram_latency "BRAM latency"
      mask TypeOptions overflow: Wrap | Saturate | Error
      mask TypeOptions quantization: Truncate | Round  (unbiased: +/- Inf) | Round  (unbiased: even values)
  quant_status : Subsystem  Tag=xps:sw_reg  AncestorBlock=xps_library/software register  mask(swreg){io_dir=To Processor, io_delay=0, sample_period=1, names=[pol0_or_cnt pol1_or_cnt], bitwidths=[6], bin_pts=0, arith_types=0, sim_port=off, show_format=on}
      mask prompts: io_dir "I/O direction"; io_delay "I/O delay"; sample_period "Sample period"; names "Bitfield names [msb...lsb]"; bitwidths "Bitfield widths"; bin_pts "Bitfield binary pts"; arith_types "Bitfield types, ufix=0, fix=1, bool=2"; sim_port "Provide sim input/output?"; show_format "Print format string?"
      mask help: A 32-bit software-accessible register. Can be divided into bitfields of varying widths and types using the fields in the block mask.
      mask init:
      | swreg_init(gcb)
      settings: AttributesFormatString=2 outputs:uf6.0,uf6.0 = 12 bits
      mask TypeOptions io_dir: To Processor | From Processor
      mask Callback io_dir:
      | mask_enables = get_param(gcb, 'MaskEnables');
      | mask_names = get_param(gcb, 'MaskNames');
      | if strcmp(get_param(gcb, 'io_dir'), 'To Processor'),
      |     mask_enables{ismember(mask_names, 'sample_period')} = 'off';
      | else
      |     mask_enables{ismember(mask_names, 'sample_period')} = 'on';
      | end
      | set_param(gcb, 'MaskEnables', mask_enables);
  reorder_status : Subsystem  Tag=xps:sw_reg  AncestorBlock=xps_library/software_register  mask(swreg){io_dir=To Processor, io_delay=0, sample_period=1, names=[timestep_err_cnt receive_err_cnt discard_cnt relock_err_cnt overflow_err_cnt dv_cnt], bitwidths=5, bin_pts=0, arith_types=0, sim_port=off, show_format=on}
      mask prompts: io_dir "I/O direction"; io_delay "I/O delay"; sample_period "Sample period"; names "Bitfield names [msb...lsb]"; bitwidths "Bitfield widths"; bin_pts "Bitfield binary pts"; arith_types "Bitfield types, ufix=0, fix=1, bool=2"; sim_port "Provide sim input/output?"; show_format "Print format string?"
      mask help: A 32-bit software-accessible register. Can be divided into bitfields of varying widths and types using the fields in the block mask.
      mask init:
      | swreg_init(gcb)
      settings: AttributesFormatString=6 outputs:uf5.0,uf5.0,uf5.0,uf5.0,uf5.0,uf5.0 = 30 bits
      mask TypeOptions io_dir: To Processor | From Processor
      mask Callback io_dir:
      | mask_enables = get_param(gcb, 'MaskEnables');
      | mask_names = get_param(gcb, 'MaskNames');
      | if strcmp(get_param(gcb, 'io_dir'), 'To Processor'),
      |     mask_enables{ismember(mask_names, 'sample_period')} = 'off';
      | else
      |     mask_enables{ismember(mask_names, 'sample_period')} = 'on';
      | end
      | set_param(gcb, 'MaskEnables', mask_enables);
  reorder_status1 : Subsystem  Tag=xps:sw_reg  AncestorBlock=xps_library/software_register  mask(swreg){io_dir=To Processor, io_delay=0, sample_period=1, names=dv_per_sec, bitwidths=32, bin_pts=0, arith_types=0, sim_port=off, show_format=on}
      mask prompts: io_dir "I/O direction"; io_delay "I/O delay"; sample_period "Sample period"; names "Bitfield names [msb...lsb]"; bitwidths "Bitfield widths"; bin_pts "Bitfield binary pts"; arith_types "Bitfield types, ufix=0, fix=1, bool=2"; sim_port "Provide sim input/output?"; show_format "Print format string?"
      mask help: A 32-bit software-accessible register. Can be divided into bitfields of varying widths and types using the fields in the block mask.
      mask init:
      | swreg_init(gcb)
      settings: AttributesFormatString=1output:uf32.0 = 32 bits
      mask TypeOptions io_dir: To Processor | From Processor
      mask Callback io_dir:
      | mask_enables = get_param(gcb, 'MaskEnables');
      | mask_names = get_param(gcb, 'MaskNames');
      | if strcmp(get_param(gcb, 'io_dir'), 'To Processor'),
      |     mask_enables{ismember(mask_names, 'sample_period')} = 'off';
      | else
      |     mask_enables{ismember(mask_names, 'sample_period')} = 'on';
      | end
      | set_param(gcb, 'MaskEnables', mask_enables);
  rx_dest_ip : Subsystem  Tag=xps:sw_reg  AncestorBlock=xps_library/software register  mask(swreg){io_dir=To Processor, io_delay=0, sample_period=1, names=reg, bitwidths=32, bin_pts=0, arith_types=0, sim_port=off, show_format=on}
      mask prompts: io_dir "I/O direction"; io_delay "I/O delay"; sample_period "Sample period"; names "Bitfield names [msb...lsb]"; bitwidths "Bitfield widths"; bin_pts "Bitfield binary pts"; arith_types "Bitfield types, ufix=0, fix=1, bool=2"; sim_port "Provide sim input/output?"; show_format "Print format string?"
      mask help: A 32-bit software-accessible register. Can be divided into bitfields of varying widths and types using the fields in the block mask.
      mask init:
      | swreg_init(gcb)
      settings: AttributesFormatString=1output:uf32.0 = 32 bits
      mask TypeOptions io_dir: To Processor | From Processor
      mask Callback io_dir:
      | mask_enables = get_param(gcb, 'MaskEnables');
      | mask_names = get_param(gcb, 'MaskNames');
      | if strcmp(get_param(gcb, 'io_dir'), 'To Processor'),
      |     mask_enables{ismember(mask_names, 'sample_period')} = 'off';
      | else
      |     mask_enables{ismember(mask_names, 'sample_period')} = 'on';
      | end
      | set_param(gcb, 'MaskEnables', mask_enables);
  rx_dest_port : Subsystem  Tag=xps:sw_reg  AncestorBlock=xps_library/software register  mask(swreg){io_dir=To Processor, io_delay=0, sample_period=1, names=reg, bitwidths=16, bin_pts=0, arith_types=0, sim_port=off, show_format=on}
      mask prompts: io_dir "I/O direction"; io_delay "I/O delay"; sample_period "Sample period"; names "Bitfield names [msb...lsb]"; bitwidths "Bitfield widths"; bin_pts "Bitfield binary pts"; arith_types "Bitfield types, ufix=0, fix=1, bool=2"; sim_port "Provide sim input/output?"; show_format "Print format string?"
      mask help: A 32-bit software-accessible register. Can be divided into bitfields of varying widths and types using the fields in the block mask.
      mask init:
      | swreg_init(gcb)
      settings: AttributesFormatString=1output:uf16.0 = 16 bits
      mask TypeOptions io_dir: To Processor | From Processor
      mask Callback io_dir:
      | mask_enables = get_param(gcb, 'MaskEnables');
      | mask_names = get_param(gcb, 'MaskNames');
      | if strcmp(get_param(gcb, 'io_dir'), 'To Processor'),
      |     mask_enables{ismember(mask_names, 'sample_period')} = 'off';
      | else
      |     mask_enables{ismember(mask_names, 'sample_period')} = 'on';
      | end
      | set_param(gcb, 'MaskEnables', mask_enables);
  rx_src_ip : Subsystem  Tag=xps:sw_reg  AncestorBlock=xps_library/software register  mask(swreg){io_dir=To Processor, io_delay=0, sample_period=1, names=reg, bitwidths=32, bin_pts=0, arith_types=0, sim_port=off, show_format=on}
      mask prompts: io_dir "I/O direction"; io_delay "I/O delay"; sample_period "Sample period"; names "Bitfield names [msb...lsb]"; bitwidths "Bitfield widths"; bin_pts "Bitfield binary pts"; arith_types "Bitfield types, ufix=0, fix=1, bool=2"; sim_port "Provide sim input/output?"; show_format "Print format string?"
      mask help: A 32-bit software-accessible register. Can be divided into bitfields of varying widths and types using the fields in the block mask.
      mask init:
      | swreg_init(gcb)
      settings: AttributesFormatString=1output:uf32.0 = 32 bits
      mask TypeOptions io_dir: To Processor | From Processor
      mask Callback io_dir:
      | mask_enables = get_param(gcb, 'MaskEnables');
      | mask_names = get_param(gcb, 'MaskNames');
      | if strcmp(get_param(gcb, 'io_dir'), 'To Processor'),
      |     mask_enables{ismember(mask_names, 'sample_period')} = 'off';
      | else
      |     mask_enables{ismember(mask_names, 'sample_period')} = 'on';
      | end
      | set_param(gcb, 'MaskEnables', mask_enables);
  rx_src_port : Subsystem  Tag=xps:sw_reg  AncestorBlock=xps_library/software register  mask(swreg){io_dir=To Processor, io_delay=0, sample_period=1, names=reg, bitwidths=16, bin_pts=0, arith_types=0, sim_port=off, show_format=on}
      mask prompts: io_dir "I/O direction"; io_delay "I/O delay"; sample_period "Sample period"; names "Bitfield names [msb...lsb]"; bitwidths "Bitfield widths"; bin_pts "Bitfield binary pts"; arith_types "Bitfield types, ufix=0, fix=1, bool=2"; sim_port "Provide sim input/output?"; show_format "Print format string?"
      mask help: A 32-bit software-accessible register. Can be divided into bitfields of varying widths and types using the fields in the block mask.
      mask init:
      | swreg_init(gcb)
      settings: AttributesFormatString=1output:uf16.0 = 16 bits
      mask TypeOptions io_dir: To Processor | From Processor
      mask Callback io_dir:
      | mask_enables = get_param(gcb, 'MaskEnables');
      | mask_names = get_param(gcb, 'MaskNames');
      | if strcmp(get_param(gcb, 'io_dir'), 'To Processor'),
      |     mask_enables{ismember(mask_names, 'sample_period')} = 'off';
      | else
      |     mask_enables{ismember(mask_names, 'sample_period')} = 'on';
      | end
      | set_param(gcb, 'MaskEnables', mask_enables);
  snap_adc0 : Subsystem  Tag=casper:bitsnap  AncestorBlock=casper_library_scopes/bitfield_snapshot  mask(bitsnap){io_names=[p0_d0 p0_d1 p0_d2 p0_d3 p0_d4 p0_d5 p0_d6 p0_d7 p1_d0 p1_d1 p1_d2 p1_d3 p1_d4_u8], io_widths=[10 10 10 10 10 10 10 10 10 10 10 10 8], io_bps=[9 9 9 9 9 9 9 9 9 9 9 9 0], io_types=[1 1 1 1 1 1 1 1 1 1 1 1 0], show_format=on, snap_storage=bram, snap_dram_dimm=2, snap_dram_clock=250, snap_nsamples=9, snap_data_width=128, snap_offset=off, snap_circap=off, snap_value=on, snap_ext_arm=off, snap_provide_outputs=on, snap_use_dsp48=on, snap_delay=2, extra_names=timestamp, extra_widths=32, extra_bps=0, extra_types=0}
      mask prompts: io_names "Names [msb...lsb]"; io_widths "Bitwidths [msb...lsb]"; io_bps "Binary pts [msb...lsb]"; io_types "Data types [msb...lsb], ufix=0, fix=1, bool=2"; show_format "Print format string?"; snap_storage "Storage medium"; snap_dram_dimm "DRAM dimm"; snap_dram_clock "DRAM clock rate"; snap_nsamples "Number of Samples (2^?)"; snap_data_width "Data width"; snap_offset "Start delay support"; snap_circap "Circular capture support"; snap_value "Extra value capture support"; snap_ext_arm "External arm support"; snap_provide_outputs "Provide outputs"; snap_use_dsp48 "Use DSP48s to implement counters"; snap_delay "Pre-snapshot delay"; extra_names "Names [msb...lsb]"; extra_widths "Widths [msb...lsb]"; extra_bps "Binary pts [msb...lsb]"; extra_types "Data types [msb...lsb], ufix=0, fix=1, bool=2"
      mask help:
      | A wrapped snapshot block. Allows specification of inputs to a snapblock word so the toolflow can automatically set up the scope.
      | See documentation for snapshot for explanation of parameters.
      mask init:
      | bitsnap_init(gcb);
      settings: AttributesFormatString=|
      | snap(13):f10.9,f10.9,f10.9,f10.9,f10.9,f10.9,f10.9,f10.9,f10.9,f10.9,f10.9,f10.9,uf8.0 = 128 bits\nextra(1):uf32.0 = 32 bits\n128 wide, 512 deep
      | debugID: 118358857
      mask TypeOptions snap_storage: bram | dram
      mask Callback snap_storage: bitsnap_callback();
      mask TypeOptions snap_dram_dimm: 1 | 2 | 3 | 4
      mask TypeOptions snap_dram_clock: 200 | 250 | 266 | 300 | 333
      mask TypeOptions snap_data_width: 8 | 16 | 32 | 64 | 128
      mask Callback snap_value: bitsnap_callback();
      mask Callback snap_ext_arm: bitsnap_callback();
      mask Callback snap_provide_outputs: bitsnap_callback();
  snap_adc1 : Subsystem  Tag=casper:bitsnap  AncestorBlock=casper_library_scopes/bitfield_snapshot  mask(bitsnap){io_names=[p1_d4_l2 p1_d5 p1_d6 p1_d7], io_widths=[2 10 10 10], io_bps=[0 9 9 9], io_types=[0 1 1 1], show_format=on, snap_storage=bram, snap_dram_dimm=2, snap_dram_clock=250, snap_nsamples=9, snap_data_width=32, snap_offset=off, snap_circap=off, snap_value=off, snap_ext_arm=off, snap_provide_outputs=on, snap_use_dsp48=on, snap_delay=2, extra_names=timestamp, extra_widths=32, extra_bps=0, extra_types=0}
      mask prompts: io_names "Names [msb...lsb]"; io_widths "Bitwidths [msb...lsb]"; io_bps "Binary pts [msb...lsb]"; io_types "Data types [msb...lsb], ufix=0, fix=1, bool=2"; show_format "Print format string?"; snap_storage "Storage medium"; snap_dram_dimm "DRAM dimm"; snap_dram_clock "DRAM clock rate"; snap_nsamples "Number of Samples (2^?)"; snap_data_width "Data width"; snap_offset "Start delay support"; snap_circap "Circular capture support"; snap_value "Extra value capture support"; snap_ext_arm "External arm support"; snap_provide_outputs "Provide outputs"; snap_use_dsp48 "Use DSP48s to implement counters"; snap_delay "Pre-snapshot delay"; extra_names "Names [msb...lsb]"; extra_widths "Widths [msb...lsb]"; extra_bps "Binary pts [msb...lsb]"; extra_types "Data types [msb...lsb], ufix=0, fix=1, bool=2"
      mask help:
      | A wrapped snapshot block. Allows specification of inputs to a snapblock word so the toolflow can automatically set up the scope.
      | See documentation for snapshot for explanation of parameters.
      mask init:
      | bitsnap_init(gcb);
      settings: AttributesFormatString=|
      | snap(4):uf2.0,f10.9,f10.9,f10.9 = 32 bits\n32 wide, 512 deep
      | debugID: 118388648
      mask TypeOptions snap_storage: bram | dram
      mask Callback snap_storage: bitsnap_callback();
      mask TypeOptions snap_dram_dimm: 1 | 2 | 3 | 4
      mask TypeOptions snap_dram_clock: 200 | 250 | 266 | 300 | 333
      mask TypeOptions snap_data_width: 8 | 16 | 32 | 64 | 128
      mask Callback snap_value: bitsnap_callback();
      mask Callback snap_ext_arm: bitsnap_callback();
      mask Callback snap_provide_outputs: bitsnap_callback();
  snap_cd_time_debug : Subsystem  Tag=casper:bitsnap  AncestorBlock=casper_library_scopes/bitfield_snapshot  mask(bitsnap){io_names=[unpack_sync unpack_dv unpack_data d80sync d80valid data80 delay_sync delay_dv delay_data cd_error0 cd_error1], io_widths=[1 1 36 1 1 36 1 1 36 1 1], io_bps=0, io_types=[2 2 0 2 2 0 2 2 0 2 2], show_format=on, snap_storage=bram, snap_dram_dimm=2, snap_dram_clock=250, snap_nsamples=13, snap_data_width=128, snap_offset=off, snap_circap=on, snap_value=off, snap_ext_arm=off, snap_provide_outputs=on, snap_use_dsp48=on, snap_delay=2, extra_names=[sync_time], extra_widths=[32], extra_bps=[0], extra_types=[0]}
      mask prompts: io_names "Names [msb...lsb]"; io_widths "Bitwidths [msb...lsb]"; io_bps "Binary pts [msb...lsb]"; io_types "Data types [msb...lsb], ufix=0, fix=1, bool=2"; show_format "Print format string?"; snap_storage "Storage medium"; snap_dram_dimm "DRAM dimm"; snap_dram_clock "DRAM clock rate"; snap_nsamples "Number of Samples (2^?)"; snap_data_width "Data width"; snap_offset "Start delay support"; snap_circap "Circular capture support"; snap_value "Extra value capture support"; snap_ext_arm "External arm support"; snap_provide_outputs "Provide outputs"; snap_use_dsp48 "Use DSP48s to implement counters"; snap_delay "Pre-snapshot delay"; extra_names "Names [msb...lsb]"; extra_widths "Widths [msb...lsb]"; extra_bps "Binary pts [msb...lsb]"; extra_types "Data types [msb...lsb], ufix=0, fix=1, bool=2"
      mask help:
      | A wrapped snapshot block. Allows specification of inputs to a snapblock word so the toolflow can automatically set up the scope.
      | See documentation for snapshot for explanation of parameters.
      mask init:
      | bitsnap_init(gcb);
      settings: AttributesFormatString=|
      | snap(11):b,b,uf36.0,b,b,uf36.0,b,b,uf36.0,b,b = 116 bits\n128 wide, 8192 deep
      | debugID: 123427494
      mask TypeOptions snap_storage: bram | dram
      mask Callback snap_storage: bitsnap_callback();
      mask TypeOptions snap_dram_dimm: 1 | 2 | 3 | 4
      mask TypeOptions snap_dram_clock: 200 | 250 | 266 | 300 | 333
      mask TypeOptions snap_data_width: 8 | 16 | 32 | 64 | 128
      mask Callback snap_value: bitsnap_callback();
      mask Callback snap_ext_arm: bitsnap_callback();
      mask Callback snap_provide_outputs: bitsnap_callback();
  snap_pre_pfb0 : Subsystem  Tag=casper:bitsnap  AncestorBlock=casper_library_scopes/bitfield_snapshot  mask(bitsnap){io_names=[d0 d1 d2 d3 d4 d5 d6 d7], io_widths=10, io_bps=9, io_types=1, show_format=on, snap_storage=bram, snap_dram_dimm=2, snap_dram_clock=250, snap_nsamples=8, snap_data_width=128, snap_offset=on, snap_circap=off, snap_value=off, snap_ext_arm=off, snap_provide_outputs=on, snap_use_dsp48=on, snap_delay=2, extra_names=[c d], extra_widths=[30 2], extra_bps=[0 0], extra_types=[0 0]}
      mask prompts: io_names "Names [msb...lsb]"; io_widths "Bitwidths [msb...lsb]"; io_bps "Binary pts [msb...lsb]"; io_types "Data types [msb...lsb], ufix=0, fix=1, bool=2"; show_format "Print format string?"; snap_storage "Storage medium"; snap_dram_dimm "DRAM dimm"; snap_dram_clock "DRAM clock rate"; snap_nsamples "Number of Samples (2^?)"; snap_data_width "Data width"; snap_offset "Start delay support"; snap_circap "Circular capture support"; snap_value "Extra value capture support"; snap_ext_arm "External arm support"; snap_provide_outputs "Provide outputs"; snap_use_dsp48 "Use DSP48s to implement counters"; snap_delay "Pre-snapshot delay"; extra_names "Names [msb...lsb]"; extra_widths "Widths [msb...lsb]"; extra_bps "Binary pts [msb...lsb]"; extra_types "Data types [msb...lsb], ufix=0, fix=1, bool=2"
      mask help:
      | A wrapped snapshot block. Allows specification of inputs to a snapblock word so the toolflow can automatically set up the scope.
      | See documentation for snapshot for explanation of parameters.
      mask init:
      | bitsnap_init(gcb);
      settings: AttributesFormatString=|
      | snap(8):f10.9,f10.9,f10.9,f10.9,f10.9,f10.9,f10.9,f10.9 = 80 bits\n128 wide, 256 deep
      | debugID: 101779257
      mask TypeOptions snap_storage: bram | dram
      mask Callback snap_storage: bitsnap_callback();
      mask TypeOptions snap_dram_dimm: 1 | 2 | 3 | 4
      mask TypeOptions snap_dram_clock: 200 | 250 | 266 | 300 | 333
      mask TypeOptions snap_data_width: 8 | 16 | 32 | 64 | 128
      mask Callback snap_value: bitsnap_callback();
      mask Callback snap_ext_arm: bitsnap_callback();
      mask Callback snap_provide_outputs: bitsnap_callback();
  snap_pre_pfb1 : Subsystem  Tag=casper:bitsnap  AncestorBlock=casper_library_scopes/bitfield_snapshot  mask(bitsnap){io_names=[d0 d1 d2 d3 d4 d5 d6 d7], io_widths=10, io_bps=9, io_types=1, show_format=on, snap_storage=bram, snap_dram_dimm=2, snap_dram_clock=250, snap_nsamples=8, snap_data_width=128, snap_offset=on, snap_circap=off, snap_value=off, snap_ext_arm=off, snap_provide_outputs=on, snap_use_dsp48=on, snap_delay=2, extra_names=[c d], extra_widths=[30 2], extra_bps=[0 0], extra_types=[0 0]}
      mask prompts: io_names "Names [msb...lsb]"; io_widths "Bitwidths [msb...lsb]"; io_bps "Binary pts [msb...lsb]"; io_types "Data types [msb...lsb], ufix=0, fix=1, bool=2"; show_format "Print format string?"; snap_storage "Storage medium"; snap_dram_dimm "DRAM dimm"; snap_dram_clock "DRAM clock rate"; snap_nsamples "Number of Samples (2^?)"; snap_data_width "Data width"; snap_offset "Start delay support"; snap_circap "Circular capture support"; snap_value "Extra value capture support"; snap_ext_arm "External arm support"; snap_provide_outputs "Provide outputs"; snap_use_dsp48 "Use DSP48s to implement counters"; snap_delay "Pre-snapshot delay"; extra_names "Names [msb...lsb]"; extra_widths "Widths [msb...lsb]"; extra_bps "Binary pts [msb...lsb]"; extra_types "Data types [msb...lsb], ufix=0, fix=1, bool=2"
      mask help:
      | A wrapped snapshot block. Allows specification of inputs to a snapblock word so the toolflow can automatically set up the scope.
      | See documentation for snapshot for explanation of parameters.
      mask init:
      | bitsnap_init(gcb);
      settings: AttributesFormatString=|
      | snap(8):f10.9,f10.9,f10.9,f10.9,f10.9,f10.9,f10.9,f10.9 = 80 bits\n128 wide, 256 deep
      | debugID: 101809048
      mask TypeOptions snap_storage: bram | dram
      mask Callback snap_storage: bitsnap_callback();
      mask TypeOptions snap_dram_dimm: 1 | 2 | 3 | 4
      mask TypeOptions snap_dram_clock: 200 | 250 | 266 | 300 | 333
      mask TypeOptions snap_data_width: 8 | 16 | 32 | 64 | 128
      mask Callback snap_value: bitsnap_callback();
      mask Callback snap_ext_arm: bitsnap_callback();
      mask Callback snap_provide_outputs: bitsnap_callback();
  snap_quant0 : Subsystem  Tag=casper:bitsnap  AncestorBlock=casper_library_scopes/bitfield_snapshot  mask(bitsnap){io_names=[real0 imag0 real1 imag1 real2 imag2 real3 imag3], io_widths=8, io_bps=7, io_types=1, show_format=on, snap_storage=bram, snap_dram_dimm=2, snap_dram_clock=250, snap_nsamples=10, snap_data_width=64, snap_offset=on, snap_circap=off, snap_value=off, snap_ext_arm=off, snap_provide_outputs=on, snap_use_dsp48=on, snap_delay=0, extra_names=[c d], extra_widths=[30 2], extra_bps=[0 0], extra_types=[0 0]}
      mask prompts: io_names "Names [msb...lsb]"; io_widths "Bitwidths [msb...lsb]"; io_bps "Binary pts [msb...lsb]"; io_types "Data types [msb...lsb], ufix=0, fix=1, bool=2"; show_format "Print format string?"; snap_storage "Storage medium"; snap_dram_dimm "DRAM dimm"; snap_dram_clock "DRAM clock rate"; snap_nsamples "Number of Samples (2^?)"; snap_data_width "Data width"; snap_offset "Start delay support"; snap_circap "Circular capture support"; snap_value "Extra value capture support"; snap_ext_arm "External arm support"; snap_provide_outputs "Provide outputs"; snap_use_dsp48 "Use DSP48s to implement counters"; snap_delay "Pre-snapshot delay"; extra_names "Names [msb...lsb]"; extra_widths "Widths [msb...lsb]"; extra_bps "Binary pts [msb...lsb]"; extra_types "Data types [msb...lsb], ufix=0, fix=1, bool=2"
      mask help:
      | A wrapped snapshot block. Allows specification of inputs to a snapblock word so the toolflow can automatically set up the scope.
      | See documentation for snapshot for explanation of parameters.
      mask init:
      | bitsnap_init(gcb);
      settings: AttributesFormatString=|
      | snap(8):f8.7,f8.7,f8.7,f8.7,f8.7,f8.7,f8.7,f8.7 = 64 bits\n64 wide, 1024 deep
      | debugID: 25309164
      mask TypeOptions snap_storage: bram | dram
      mask Callback snap_storage: bitsnap_callback();
      mask TypeOptions snap_dram_dimm: 1 | 2 | 3 | 4
      mask TypeOptions snap_dram_clock: 200 | 250 | 266 | 300 | 333
      mask TypeOptions snap_data_width: 8 | 16 | 32 | 64 | 128
      mask Callback snap_value: bitsnap_callback();
      mask Callback snap_ext_arm: bitsnap_callback();
      mask Callback snap_provide_outputs: bitsnap_callback();
  snap_quant1 : Subsystem  Tag=casper:bitsnap  AncestorBlock=casper_library_scopes/bitfield_snapshot  mask(bitsnap){io_names=[real0 imag0 real1 imag1 real2 imag2 real3 imag3], io_widths=8, io_bps=7, io_types=1, show_format=on, snap_storage=bram, snap_dram_dimm=2, snap_dram_clock=250, snap_nsamples=10, snap_data_width=64, snap_offset=on, snap_circap=off, snap_value=off, snap_ext_arm=off, snap_provide_outputs=on, snap_use_dsp48=on, snap_delay=0, extra_names=[c d], extra_widths=[30 2], extra_bps=[0 0], extra_types=[0 0]}
      mask prompts: io_names "Names [msb...lsb]"; io_widths "Bitwidths [msb...lsb]"; io_bps "Binary pts [msb...lsb]"; io_types "Data types [msb...lsb], ufix=0, fix=1, bool=2"; show_format "Print format string?"; snap_storage "Storage medium"; snap_dram_dimm "DRAM dimm"; snap_dram_clock "DRAM clock rate"; snap_nsamples "Number of Samples (2^?)"; snap_data_width "Data width"; snap_offset "Start delay support"; snap_circap "Circular capture support"; snap_value "Extra value capture support"; snap_ext_arm "External arm support"; snap_provide_outputs "Provide outputs"; snap_use_dsp48 "Use DSP48s to implement counters"; snap_delay "Pre-snapshot delay"; extra_names "Names [msb...lsb]"; extra_widths "Widths [msb...lsb]"; extra_bps "Binary pts [msb...lsb]"; extra_types "Data types [msb...lsb], ufix=0, fix=1, bool=2"
      mask help:
      | A wrapped snapshot block. Allows specification of inputs to a snapblock word so the toolflow can automatically set up the scope.
      | See documentation for snapshot for explanation of parameters.
      mask init:
      | bitsnap_init(gcb);
      settings: AttributesFormatString=|
      | snap(8):f8.7,f8.7,f8.7,f8.7,f8.7,f8.7,f8.7,f8.7 = 64 bits\n64 wide, 1024 deep
      | debugID: 25338955
      mask TypeOptions snap_storage: bram | dram
      mask Callback snap_storage: bitsnap_callback();
      mask TypeOptions snap_dram_dimm: 1 | 2 | 3 | 4
      mask TypeOptions snap_dram_clock: 200 | 250 | 266 | 300 | 333
      mask TypeOptions snap_data_width: 8 | 16 | 32 | 64 | 128
      mask Callback snap_value: bitsnap_callback();
      mask Callback snap_ext_arm: bitsnap_callback();
      mask Callback snap_provide_outputs: bitsnap_callback();
  spead_status : Subsystem  Tag=xps:sw_reg  AncestorBlock=xps_library/software_register  mask(swreg){io_dir=To Processor, io_delay=0, sample_period=1, names=[magic_err_cnt header_err_cnt pad_err_cnt pkt_len_err_cnt pkt_cnt], bitwidths=6, bin_pts=0, arith_types=0, sim_port=off, show_format=on}
      mask prompts: io_dir "I/O direction"; io_delay "I/O delay"; sample_period "Sample period"; names "Bitfield names [msb...lsb]"; bitwidths "Bitfield widths"; bin_pts "Bitfield binary pts"; arith_types "Bitfield types, ufix=0, fix=1, bool=2"; sim_port "Provide sim input/output?"; show_format "Print format string?"
      mask help: A 32-bit software-accessible register. Can be divided into bitfields of varying widths and types using the fields in the block mask.
      mask init:
      | swreg_init(gcb)
      settings: AttributesFormatString=5 outputs:uf6.0,uf6.0,uf6.0,uf6.0,uf6.0 = 30 bits
      mask TypeOptions io_dir: To Processor | From Processor
      mask Callback io_dir:
      | mask_enables = get_param(gcb, 'MaskEnables');
      | mask_names = get_param(gcb, 'MaskNames');
      | if strcmp(get_param(gcb, 'io_dir'), 'To Processor'),
      |     mask_enables{ismember(mask_names, 'sample_period')} = 'off';
      | else
      |     mask_enables{ismember(mask_names, 'sample_period')} = 'on';
      | end
      | set_param(gcb, 'MaskEnables', mask_enables);
  sync80_count : Subsystem  Tag=xps:sw_reg  AncestorBlock=xps_library/software_register  mask(swreg){io_dir=To Processor, io_delay=0, sample_period=1, names=reg, bitwidths=32, bin_pts=0, arith_types=0, sim_port=off, show_format=on}
      mask prompts: io_dir "I/O direction"; io_delay "I/O delay"; sample_period "Sample period"; names "Bitfield names [msb...lsb]"; bitwidths "Bitfield widths"; bin_pts "Bitfield binary pts"; arith_types "Bitfield types, ufix=0, fix=1, bool=2"; sim_port "Provide sim input/output?"; show_format "Print format string?"
      mask help: A 32-bit software-accessible register. Can be divided into bitfields of varying widths and types using the fields in the block mask.
      mask init:
      | swreg_init(gcb)
      settings: AttributesFormatString=1output:uf32.0 = 32 bits
      mask TypeOptions io_dir: To Processor | From Processor
      mask Callback io_dir:
      | mask_enables = get_param(gcb, 'MaskEnables');
      | mask_names = get_param(gcb, 'MaskNames');
      | if strcmp(get_param(gcb, 'io_dir'), 'To Processor'),
      |     mask_enables{ismember(mask_names, 'sample_period')} = 'off';
      | else
      |     mask_enables{ismember(mask_names, 'sample_period')} = 'on';
      | end
      | set_param(gcb, 'MaskEnables', mask_enables);
  sync_gen : Subsystem  mask{zerolsbs=24}
      mask prompts: zerolsbs "No. LSBs to be zero:"
  time_gen : Subsystem  mask{n_bits_period=fft_stages-1-2, n_bits_increment=0, n_bits_counter=48-fft_stages}
      mask prompts: n_bits_period "Period (2^?)"; n_bits_increment "Increment (2^?)"; n_bits_counter "Counter size (2^?)"
  time_gen1 : Subsystem  mask{n_bits_period=fft_stages-1-2-1+8, n_bits_increment=0, n_bits_counter=48-(fft_stages+8)}
      mask prompts: n_bits_period "Period (2^?)"; n_bits_increment "Increment (2^?)"; n_bits_counter "Counter size (2^?)"
  time_gen_cd : Subsystem  mask{n_bits_period=fft_stages-1-2, n_bits_increment=0, n_bits_counter=48-fft_stages}
      mask prompts: n_bits_period "Period (2^?)"; n_bits_increment "Increment (2^?)"; n_bits_counter "Counter size (2^?)"
  time_status : Subsystem  Tag=xps:sw_reg  AncestorBlock=xps_library/software_register  mask(swreg){io_dir=To Processor, io_delay=0, sample_period=1, names=dv_cnt, bitwidths=32, bin_pts=0, arith_types=0, sim_port=off, show_format=on}
      mask prompts: io_dir "I/O direction"; io_delay "I/O delay"; sample_period "Sample period"; names "Bitfield names [msb...lsb]"; bitwidths "Bitfield widths"; bin_pts "Bitfield binary pts"; arith_types "Bitfield types, ufix=0, fix=1, bool=2"; sim_port "Provide sim input/output?"; show_format "Print format string?"
      mask help: A 32-bit software-accessible register. Can be divided into bitfields of varying widths and types using the fields in the block mask.
      mask init:
      | swreg_init(gcb)
      settings: AttributesFormatString=1output:uf32.0 = 32 bits
      mask TypeOptions io_dir: To Processor | From Processor
      mask Callback io_dir:
      | mask_enables = get_param(gcb, 'MaskEnables');
      | mask_names = get_param(gcb, 'MaskNames');
      | if strcmp(get_param(gcb, 'io_dir'), 'To Processor'),
      |     mask_enables{ismember(mask_names, 'sample_period')} = 'off';
      | else
      |     mask_enables{ismember(mask_names, 'sample_period')} = 'on';
      | end
      | set_param(gcb, 'MaskEnables', mask_enables);
  tl_cd0 : Subsystem  mask(timed_latch){n_bits_time=48-fft_stages, n_bits_quantization=fft_stages, n_bits_counters=4}
      mask prompts: n_bits_time "Number bits in time to compare"; n_bits_quantization "Time offset from lsb"; n_bits_counters "Bits in status counters"
      mask help:
      | Latches load_value when armed and current_time matches requested time.
      | current_time should be in ADC samples.
      mask init:
      | set_param([gcb,'/status'], 'bitwidths', mat2str([1, repmat(n_bits_counters, 1, 2)]));
      mask Help:
      | When armed, will latch new value when current time matches the time
      | specified. The input time should be in samples and mask settings allow
      | a portion of this to be compared to cater for quantization. Arm and latch
      | counts allow the current state, pending and missed latch events to be
      | determined.
  tl_cd0_control : Subsystem  Tag=xps:sw_reg  AncestorBlock=xps_library/software_register  mask(swreg){io_dir=From Processor, io_delay=0, sample_period=1, names=load_time_lsw, bitwidths=32, bin_pts=0, arith_types=0, sim_port=on, show_format=on}
      mask prompts: io_dir "I/O direction"; io_delay "I/O delay"; sample_period "Sample period"; names "Bitfield names [msb...lsb]"; bitwidths "Bitfield widths"; bin_pts "Bitfield binary pts"; arith_types "Bitfield types, ufix=0, fix=1, bool=2"; sim_port "Provide sim input/output?"; show_format "Print format string?"
      mask help: A 32-bit software-accessible register. Can be divided into bitfields of varying widths and types using the fields in the block mask.
      mask init:
      | swreg_init(gcb)
      settings: AttributesFormatString=1input:uf32.0 = 32 bits
      mask TypeOptions io_dir: To Processor | From Processor
      mask Callback io_dir:
      | mask_enables = get_param(gcb, 'MaskEnables');
      | mask_names = get_param(gcb, 'MaskNames');
      | if strcmp(get_param(gcb, 'io_dir'), 'To Processor'),
      |     mask_enables{ismember(mask_names, 'sample_period')} = 'off';
      | else
      |     mask_enables{ismember(mask_names, 'sample_period')} = 'on';
      | end
      | set_param(gcb, 'MaskEnables', mask_enables);
  tl_cd0_control0 : Subsystem  Tag=xps:sw_reg  AncestorBlock=xps_library/software_register  mask(swreg){io_dir=From Processor, io_delay=0, sample_period=1, names=[arm load_immediate load_time_msw], bitwidths=[1 1 16], bin_pts=[0 0 0], arith_types=[2 2 0], sim_port=on, show_format=on}
      mask prompts: io_dir "I/O direction"; io_delay "I/O delay"; sample_period "Sample period"; names "Bitfield names [msb...lsb]"; bitwidths "Bitfield widths"; bin_pts "Bitfield binary pts"; arith_types "Bitfield types, ufix=0, fix=1, bool=2"; sim_port "Provide sim input/output?"; show_format "Print format string?"
      mask help: A 32-bit software-accessible register. Can be divided into bitfields of varying widths and types using the fields in the block mask.
      mask init:
      | swreg_init(gcb)
      settings: AttributesFormatString=3 inputs:b,b,uf16.0 = 18 bits
      mask TypeOptions io_dir: To Processor | From Processor
      mask Callback io_dir:
      | mask_enables = get_param(gcb, 'MaskEnables');
      | mask_names = get_param(gcb, 'MaskNames');
      | if strcmp(get_param(gcb, 'io_dir'), 'To Processor'),
      |     mask_enables{ismember(mask_names, 'sample_period')} = 'off';
      | else
      |     mask_enables{ismember(mask_names, 'sample_period')} = 'on';
      | end
      | set_param(gcb, 'MaskEnables', mask_enables);
  tl_cd1 : Subsystem  mask(timed_latch){n_bits_time=48-fft_stages, n_bits_quantization=fft_stages, n_bits_counters=4}
      mask prompts: n_bits_time "Number bits in time to compare"; n_bits_quantization "Time offset from lsb"; n_bits_counters "Bits in status counters"
      mask help:
      | Latches load_value when armed and current_time matches requested time.
      | current_time should be in ADC samples.
      mask init:
      | set_param([gcb,'/status'], 'bitwidths', mat2str([1, repmat(n_bits_counters, 1, 2)]));
      mask Help:
      | When armed, will latch new value when current time matches the time
      | specified. The input time should be in samples and mask settings allow
      | a portion of this to be compared to cater for quantization. Arm and latch
      | counts allow the current state, pending and missed latch events to be
      | determined.
  tl_cd1_control : Subsystem  Tag=xps:sw_reg  AncestorBlock=xps_library/software_register  mask(swreg){io_dir=From Processor, io_delay=0, sample_period=1, names=load_time_lsw, bitwidths=32, bin_pts=0, arith_types=0, sim_port=on, show_format=on}
      mask prompts: io_dir "I/O direction"; io_delay "I/O delay"; sample_period "Sample period"; names "Bitfield names [msb...lsb]"; bitwidths "Bitfield widths"; bin_pts "Bitfield binary pts"; arith_types "Bitfield types, ufix=0, fix=1, bool=2"; sim_port "Provide sim input/output?"; show_format "Print format string?"
      mask help: A 32-bit software-accessible register. Can be divided into bitfields of varying widths and types using the fields in the block mask.
      mask init:
      | swreg_init(gcb)
      settings: AttributesFormatString=1input:uf32.0 = 32 bits
      mask TypeOptions io_dir: To Processor | From Processor
      mask Callback io_dir:
      | mask_enables = get_param(gcb, 'MaskEnables');
      | mask_names = get_param(gcb, 'MaskNames');
      | if strcmp(get_param(gcb, 'io_dir'), 'To Processor'),
      |     mask_enables{ismember(mask_names, 'sample_period')} = 'off';
      | else
      |     mask_enables{ismember(mask_names, 'sample_period')} = 'on';
      | end
      | set_param(gcb, 'MaskEnables', mask_enables);
  tl_cd1_control0 : Subsystem  Tag=xps:sw_reg  AncestorBlock=xps_library/software_register  mask(swreg){io_dir=From Processor, io_delay=0, sample_period=1, names=[arm load_immediate load_time_msw], bitwidths=[1 1 16], bin_pts=[0 0 0], arith_types=[2 2 0], sim_port=on, show_format=on}
      mask prompts: io_dir "I/O direction"; io_delay "I/O delay"; sample_period "Sample period"; names "Bitfield names [msb...lsb]"; bitwidths "Bitfield widths"; bin_pts "Bitfield binary pts"; arith_types "Bitfield types, ufix=0, fix=1, bool=2"; sim_port "Provide sim input/output?"; show_format "Print format string?"
      mask help: A 32-bit software-accessible register. Can be divided into bitfields of varying widths and types using the fields in the block mask.
      mask init:
      | swreg_init(gcb)
      settings: AttributesFormatString=3 inputs:b,b,uf16.0 = 18 bits
      mask TypeOptions io_dir: To Processor | From Processor
      mask Callback io_dir:
      | mask_enables = get_param(gcb, 'MaskEnables');
      | mask_names = get_param(gcb, 'MaskNames');
      | if strcmp(get_param(gcb, 'io_dir'), 'To Processor'),
      |     mask_enables{ismember(mask_names, 'sample_period')} = 'off';
      | else
      |     mask_enables{ismember(mask_names, 'sample_period')} = 'on';
      | end
      | set_param(gcb, 'MaskEnables', mask_enables);
  tl_cd_bs0 : Subsystem  mask(timed_latch){n_bits_time=48-fft_stages, n_bits_quantization=fft_stages, n_bits_counters=4}
      mask prompts: n_bits_time "Number bits in time to compare"; n_bits_quantization "Time offset from lsb"; n_bits_counters "Bits in status counters"
      mask help:
      | Latches load_value when armed and current_time matches requested time.
      | current_time should be in ADC samples.
      mask init:
      | set_param([gcb,'/status'], 'bitwidths', mat2str([1, repmat(n_bits_counters, 1, 2)]));
      mask Help:
      | When armed, will latch new value when current time matches the time
      | specified. The input time should be in samples and mask settings allow
      | a portion of this to be compared to cater for quantization. Arm and latch
      | counts allow the current state, pending and missed latch events to be
      | determined.
  tl_cd_bs1 : Subsystem  mask(timed_latch){n_bits_time=48-fft_stages, n_bits_quantization=fft_stages, n_bits_counters=4}
      mask prompts: n_bits_time "Number bits in time to compare"; n_bits_quantization "Time offset from lsb"; n_bits_counters "Bits in status counters"
      mask help:
      | Latches load_value when armed and current_time matches requested time.
      | current_time should be in ADC samples.
      mask init:
      | set_param([gcb,'/status'], 'bitwidths', mat2str([1, repmat(n_bits_counters, 1, 2)]));
      mask Help:
      | When armed, will latch new value when current time matches the time
      | specified. The input time should be in samples and mask settings allow
      | a portion of this to be compared to cater for quantization. Arm and latch
      | counts allow the current state, pending and missed latch events to be
      | determined.
  tl_fd0 : Subsystem  mask(timed_latch){n_bits_time=48-fft_stages, n_bits_quantization=fft_stages, n_bits_counters=4}
      mask prompts: n_bits_time "Number bits in time to compare"; n_bits_quantization "Time offset from lsb"; n_bits_counters "Bits in status counters"
      mask help:
      | Latches load_value when armed and current_time matches requested time.
      | current_time should be in ADC samples.
      mask init:
      | set_param([gcb,'/status'], 'bitwidths', mat2str([1, repmat(n_bits_counters, 1, 2)]));
      mask Help:
      | When armed, will latch new value when current time matches the time
      | specified. The input time should be in samples and mask settings allow
      | a portion of this to be compared to cater for quantization. Arm and latch
      | counts allow the current state, pending and missed latch events to be
      | determined.
  tl_fd1 : Subsystem  mask(timed_latch){n_bits_time=48-fft_stages, n_bits_quantization=fft_stages, n_bits_counters=4}
      mask prompts: n_bits_time "Number bits in time to compare"; n_bits_quantization "Time offset from lsb"; n_bits_counters "Bits in status counters"
      mask help:
      | Latches load_value when armed and current_time matches requested time.
      | current_time should be in ADC samples.
      mask init:
      | set_param([gcb,'/status'], 'bitwidths', mat2str([1, repmat(n_bits_counters, 1, 2)]));
      mask Help:
      | When armed, will latch new value when current time matches the time
      | specified. The input time should be in samples and mask settings allow
      | a portion of this to be compared to cater for quantization. Arm and latch
      | counts allow the current state, pending and missed latch events to be
      | determined.
  trig_time_lsw : Subsystem  Tag=xps:sw_reg  AncestorBlock=xps_library/software register  mask(swreg){io_dir=From Processor, io_delay=0, sample_period=1, names=lsw, bitwidths=32, bin_pts=0, arith_types=0, sim_port=off, show_format=on}
      mask prompts: io_dir "I/O direction"; io_delay "I/O delay"; sample_period "Sample period"; names "Bitfield names [msb...lsb]"; bitwidths "Bitfield widths"; bin_pts "Bitfield binary pts"; arith_types "Bitfield types, ufix=0, fix=1, bool=2"; sim_port "Provide sim input/output?"; show_format "Print format string?"
      mask help: A 32-bit software-accessible register. Can be divided into bitfields of varying widths and types using the fields in the block mask.
      mask init:
      | swreg_init(gcb)
      settings: AttributesFormatString=1input:uf32.0 = 32 bits
      mask TypeOptions io_dir: To Processor | From Processor
      mask Callback io_dir:
      | mask_enables = get_param(gcb, 'MaskEnables');
      | mask_names = get_param(gcb, 'MaskNames');
      | if strcmp(get_param(gcb, 'io_dir'), 'To Processor'),
      |     mask_enables{ismember(mask_names, 'sample_period')} = 'off';
      | else
      |     mask_enables{ismember(mask_names, 'sample_period')} = 'on';
      | end
      | set_param(gcb, 'MaskEnables', mask_enables);
  trig_time_msw : Subsystem  Tag=xps:sw_reg  AncestorBlock=xps_library/software register  mask(swreg){io_dir=From Processor, io_delay=0, sample_period=1, names=msw, bitwidths=16, bin_pts=0, arith_types=0, sim_port=off, show_format=on}
      mask prompts: io_dir "I/O direction"; io_delay "I/O delay"; sample_period "Sample period"; names "Bitfield names [msb...lsb]"; bitwidths "Bitfield widths"; bin_pts "Bitfield binary pts"; arith_types "Bitfield types, ufix=0, fix=1, bool=2"; sim_port "Provide sim input/output?"; show_format "Print format string?"
      mask help: A 32-bit software-accessible register. Can be divided into bitfields of varying widths and types using the fields in the block mask.
      mask init:
      | swreg_init(gcb)
      settings: AttributesFormatString=1input:uf16.0 = 16 bits
      mask TypeOptions io_dir: To Processor | From Processor
      mask Callback io_dir:
      | mask_enables = get_param(gcb, 'MaskEnables');
      | mask_names = get_param(gcb, 'MaskNames');
      | if strcmp(get_param(gcb, 'io_dir'), 'To Processor'),
      |     mask_enables{ismember(mask_names, 'sample_period')} = 'off';
      | else
      |     mask_enables{ismember(mask_names, 'sample_period')} = 'on';
      | end
      | set_param(gcb, 'MaskEnables', mask_enables);
  ts_tvg : Subsystem
  tvg : Subsystem
  tvg_tone_levels : Subsystem  Tag=xps:sw_reg  AncestorBlock=xps_library/software_register  mask(swreg){io_dir=From Processor, io_delay=0, sample_period=1, names=[p0r p0i p1r p1i], bitwidths=8, bin_pts=7, arith_types=1, sim_port=on, show_format=on}
      mask prompts: io_dir "I/O direction"; io_delay "I/O delay"; sample_period "Sample period"; names "Bitfield names [msb...lsb]"; bitwidths "Bitfield widths"; bin_pts "Bitfield binary pts"; arith_types "Bitfield types, ufix=0, fix=1, bool=2"; sim_port "Provide sim input/output?"; show_format "Print format string?"
      mask help: A 32-bit software-accessible register. Can be divided into bitfields of varying widths and types using the fields in the block mask.
      mask init:
      | swreg_init(gcb)
      settings: AttributesFormatString=4 inputs:f8.7,f8.7,f8.7,f8.7 = 32 bits
      mask TypeOptions io_dir: To Processor | From Processor
      mask Callback io_dir:
      | mask_enables = get_param(gcb, 'MaskEnables');
      | mask_names = get_param(gcb, 'MaskNames');
      | if strcmp(get_param(gcb, 'io_dir'), 'To Processor'),
      |     mask_enables{ismember(mask_names, 'sample_period')} = 'off';
      | else
      |     mask_enables{ismember(mask_names, 'sample_period')} = 'on';
      | end
      | set_param(gcb, 'MaskEnables', mask_enables);
  tvg_tone_targets : Subsystem  Tag=xps:sw_reg  AncestorBlock=xps_library/software_register  mask(swreg){io_dir=From Processor, io_delay=0, sample_period=1, names=[p0 p1], bitwidths=12, bin_pts=0, arith_types=0, sim_port=on, show_format=on}
      mask prompts: io_dir "I/O direction"; io_delay "I/O delay"; sample_period "Sample period"; names "Bitfield names [msb...lsb]"; bitwidths "Bitfield widths"; bin_pts "Bitfield binary pts"; arith_types "Bitfield types, ufix=0, fix=1, bool=2"; sim_port "Provide sim input/output?"; show_format "Print format string?"
      mask help: A 32-bit software-accessible register. Can be divided into bitfields of varying widths and types using the fields in the block mask.
      mask init:
      | swreg_init(gcb)
      settings: AttributesFormatString=2 inputs:uf12.0,uf12.0 = 24 bits
      mask TypeOptions io_dir: To Processor | From Processor
      mask Callback io_dir:
      | mask_enables = get_param(gcb, 'MaskEnables');
      | mask_names = get_param(gcb, 'MaskNames');
      | if strcmp(get_param(gcb, 'io_dir'), 'To Processor'),
      |     mask_enables{ismember(mask_names, 'sample_period')} = 'off';
      | else
      |     mask_enables{ismember(mask_names, 'sample_period')} = 'on';
      | end
      | set_param(gcb, 'MaskEnables', mask_enables);
  tx_metadata : Subsystem  Tag=xps:sw_reg  AncestorBlock=xps_library/software register  mask(swreg){io_dir=From Processor, io_delay=0, sample_period=1, names=[porttx board_id], bitwidths=16, bin_pts=0, arith_types=0, sim_port=off, show_format=on}
      mask prompts: io_dir "I/O direction"; io_delay "I/O delay"; sample_period "Sample period"; names "Bitfield names [msb...lsb]"; bitwidths "Bitfield widths"; bin_pts "Bitfield binary pts"; arith_types "Bitfield types, ufix=0, fix=1, bool=2"; sim_port "Provide sim input/output?"; show_format "Print format string?"
      mask help: A 32-bit software-accessible register. Can be divided into bitfields of varying widths and types using the fields in the block mask.
      mask init:
      | swreg_init(gcb)
      settings: AttributesFormatString=2 inputs:uf16.0,uf16.0 = 32 bits
      mask TypeOptions io_dir: To Processor | From Processor
      mask Callback io_dir:
      | mask_enables = get_param(gcb, 'MaskEnables');
      | mask_names = get_param(gcb, 'MaskNames');
      | if strcmp(get_param(gcb, 'io_dir'), 'To Processor'),
      |     mask_enables{ismember(mask_names, 'sample_period')} = 'off';
      | else
      |     mask_enables{ismember(mask_names, 'sample_period')} = 'on';
      | end
      | set_param(gcb, 'MaskEnables', mask_enables);
  unpack_and_reorder : Subsystem
  wb_prog_delay : Subsystem  mask{n_bits_fft=fft_stages, n_bits_cd=17}
      mask prompts: n_bits_fft "fft length (2^?)"; n_bits_cd "max coarse delay (2^?)"
  wb_prog_delay1 : Subsystem  mask{n_bits_fft=fft_stages, n_bits_cd=17}
      mask prompts: n_bits_fft "fft length (2^?)"; n_bits_cd "max coarse delay (2^?)"
  we_delay1 : Subsystem  AncestorBlock=casper_library_delays/pipeline  mask(pipeline){latency=2}
      mask help:
      | An explicitly laid-out delay line to avoid mapping to SRL16s
      | for use in pipelining to help achieve timing closure.
      mask init:
      | pipeline_init(gcb,'latency',latency);
      settings: AttributesFormatString=Latency = %<latency>
      mask Display:
      | port_label('input', 1, 'd');
      | port_label('output', 1, 'q');
      | disp(['Z^-', num2str(latency)]);
  we_delay13 : Subsystem  AncestorBlock=casper_library_delays/pipeline  mask(pipeline){latency=2}
      mask help:
      | An explicitly laid-out delay line to avoid mapping to SRL16s
      | for use in pipelining to help achieve timing closure.
      mask init:
      | pipeline_init(gcb,'latency',latency);
      settings: AttributesFormatString=Latency = %<latency>
      mask Display:
      | port_label('input', 1, 'd');
      | port_label('output', 1, 'q');
      | disp(['Z^-', num2str(latency)]);
  we_delay2 : Subsystem  AncestorBlock=casper_library_delays/pipeline  mask(pipeline){latency=2}
      mask help:
      | An explicitly laid-out delay line to avoid mapping to SRL16s
      | for use in pipelining to help achieve timing closure.
      mask init:
      | pipeline_init(gcb,'latency',latency);
      settings: AttributesFormatString=Latency = %<latency>
      mask Display:
      | port_label('input', 1, 'd');
      | port_label('output', 1, 'q');
      | disp(['Z^-', num2str(latency)]);
  we_delay29 : Subsystem  AncestorBlock=casper_library_delays/pipeline  mask(pipeline){latency=2}
      mask help:
      | An explicitly laid-out delay line to avoid mapping to SRL16s
      | for use in pipelining to help achieve timing closure.
      mask init:
      | pipeline_init(gcb,'latency',latency);
      settings: AttributesFormatString=Latency = %<latency>
      mask Display:
      | port_label('input', 1, 'd');
      | port_label('output', 1, 'q');
      | disp(['Z^-', num2str(latency)]);
  we_delay37 : Subsystem  AncestorBlock=casper_library_delays/pipeline  mask(pipeline){latency=2}
      mask help:
      | An explicitly laid-out delay line to avoid mapping to SRL16s
      | for use in pipelining to help achieve timing closure.
      mask init:
      | pipeline_init(gcb,'latency',latency);
      settings: AttributesFormatString=Latency = %<latency>
      mask Display:
      | port_label('input', 1, 'd');
      | port_label('output', 1, 'q');
      | disp(['Z^-', num2str(latency)]);
  we_delay38 : Subsystem  AncestorBlock=casper_library_delays/pipeline  mask(pipeline){latency=2}
      mask help:
      | An explicitly laid-out delay line to avoid mapping to SRL16s
      | for use in pipelining to help achieve timing closure.
      mask init:
      | pipeline_init(gcb,'latency',latency);
      settings: AttributesFormatString=Latency = %<latency>
      mask Display:
      | port_label('input', 1, 'd');
      | port_label('output', 1, 'q');
      | disp(['Z^-', num2str(latency)]);
  we_delay39 : Subsystem  AncestorBlock=casper_library_delays/pipeline  mask(pipeline){latency=2}
      mask help:
      | An explicitly laid-out delay line to avoid mapping to SRL16s
      | for use in pipelining to help achieve timing closure.
      mask init:
      | pipeline_init(gcb,'latency',latency);
      settings: AttributesFormatString=Latency = %<latency>
      mask Display:
      | port_label('input', 1, 'd');
      | port_label('output', 1, 'q');
      | disp(['Z^-', num2str(latency)]);
  we_delay45 : Subsystem  AncestorBlock=casper_library_delays/pipeline  mask(pipeline){latency=2}
      mask help:
      | An explicitly laid-out delay line to avoid mapping to SRL16s
      | for use in pipelining to help achieve timing closure.
      mask init:
      | pipeline_init(gcb,'latency',latency);
      settings: AttributesFormatString=Latency = %<latency>
      mask Display:
      | port_label('input', 1, 'd');
      | port_label('output', 1, 'q');
      | disp(['Z^-', num2str(latency)]);
  we_delay46 : Subsystem  AncestorBlock=casper_library_delays/pipeline  mask(pipeline){latency=2}
      mask help:
      | An explicitly laid-out delay line to avoid mapping to SRL16s
      | for use in pipelining to help achieve timing closure.
      mask init:
      | pipeline_init(gcb,'latency',latency);
      settings: AttributesFormatString=Latency = %<latency>
      mask Display:
      | port_label('input', 1, 'd');
      | port_label('output', 1, 'q');
      | disp(['Z^-', num2str(latency)]);
  we_delay47 : Subsystem  AncestorBlock=casper_library_delays/pipeline  mask(pipeline){latency=2}
      mask help:
      | An explicitly laid-out delay line to avoid mapping to SRL16s
      | for use in pipelining to help achieve timing closure.
      mask init:
      | pipeline_init(gcb,'latency',latency);
      settings: AttributesFormatString=Latency = %<latency>
      mask Display:
      | port_label('input', 1, 'd');
      | port_label('output', 1, 'q');
      | disp(['Z^-', num2str(latency)]);
  we_delay48 : Subsystem  AncestorBlock=casper_library_delays/pipeline  mask(pipeline){latency=2}
      mask help:
      | An explicitly laid-out delay line to avoid mapping to SRL16s
      | for use in pipelining to help achieve timing closure.
      mask init:
      | pipeline_init(gcb,'latency',latency);
      settings: AttributesFormatString=Latency = %<latency>
      mask Display:
      | port_label('input', 1, 'd');
      | port_label('output', 1, 'q');
      | disp(['Z^-', num2str(latency)]);
  we_delay49 : Subsystem  AncestorBlock=casper_library_delays/pipeline  mask(pipeline){latency=2}
      mask help:
      | An explicitly laid-out delay line to avoid mapping to SRL16s
      | for use in pipelining to help achieve timing closure.
      mask init:
      | pipeline_init(gcb,'latency',latency);
      settings: AttributesFormatString=Latency = %<latency>
      mask Display:
      | port_label('input', 1, 'd');
      | port_label('output', 1, 'q');
      | disp(['Z^-', num2str(latency)]);
  we_delay50 : Subsystem  AncestorBlock=casper_library_delays/pipeline  mask(pipeline){latency=2}
      mask help:
      | An explicitly laid-out delay line to avoid mapping to SRL16s
      | for use in pipelining to help achieve timing closure.
      mask init:
      | pipeline_init(gcb,'latency',latency);
      settings: AttributesFormatString=Latency = %<latency>
      mask Display:
      | port_label('input', 1, 'd');
      | port_label('output', 1, 'q');
      | disp(['Z^-', num2str(latency)]);
  we_delay7 : Subsystem  AncestorBlock=casper_library_delays/pipeline  mask(pipeline){latency=2}
      mask help:
      | An explicitly laid-out delay line to avoid mapping to SRL16s
      | for use in pipelining to help achieve timing closure.
      mask init:
      | pipeline_init(gcb,'latency',latency);
      settings: AttributesFormatString=Latency = %<latency>
      mask Display:
      | port_label('input', 1, 'd');
      | port_label('output', 1, 'q');
      | disp(['Z^-', num2str(latency)]);
  x_setup : Subsystem  Tag=xps:sw_reg  AncestorBlock=xps_library/software_register  mask(swreg){io_dir=From Processor, io_delay=0, sample_period=1, names=[f_per_x ip_per_x num_x snap_arm pktstart_mux pack_mux pktoffset_sel], bitwidths=[15 4 9 1 1 1 1], bin_pts=[0 2 0 0 0 0 0], arith_types=[0 0 0 2 0 2 0], sim_port=off, show_format=on}
      mask prompts: io_dir "I/O direction"; io_delay "I/O delay"; sample_period "Sample period"; names "Bitfield names [msb...lsb]"; bitwidths "Bitfield widths"; bin_pts "Bitfield binary pts"; arith_types "Bitfield types, ufix=0, fix=1, bool=2"; sim_port "Provide sim input/output?"; show_format "Print format string?"
      mask help: A 32-bit software-accessible register. Can be divided into bitfields of varying widths and types using the fields in the block mask.
      mask init:
      | swreg_init(gcb)
      settings: AttributesFormatString=7 inputs:uf15.0,uf4.2,uf9.0,b,uf1.0,b,uf1.0 = 32 bits
      mask TypeOptions io_dir: To Processor | From Processor
      mask Callback io_dir:
      | mask_enables = get_param(gcb, 'MaskEnables');
      | mask_names = get_param(gcb, 'MaskNames');
      | if strcmp(get_param(gcb, 'io_dir'), 'To Processor'),
      |     mask_enables{ismember(mask_names, 'sample_period')} = 'off';
      | else
      |     mask_enables{ismember(mask_names, 'sample_period')} = 'on';
      | end
      | set_param(gcb, 'MaskEnables', mask_enables);
      mask DialogControl ParameterTabVar0 Prompt: Setup
  xsg_core_config : Subsystem  Tag=xps:xsg  AncestorBlock=xps_library/XSG_core_config  mask(xsg core config){hw_sys=SKARAB:xc7vx690t, clk_src=sys_clk, clk_rate=238, sample_period=1, synthesis_tool=XST}
      mask prompts: hw_sys "Hardware Platform"; clk_src "User IP Clock source"; clk_rate "User IP Clock Rate (MHz)"; sample_period "Sample Period"; synthesis_tool "Synthesis Tool:"
      mask help:
      | The XSG Core Config block is used to configure the System Generator design
      | for the casper_xps toolflow. Settings here are used to configure the
      | Xilinx System Generator block parameters automatically, and control toolflow
      | script  execution. It needs to be at the top level of all designs being compiled
      | with the casper_xps toolflow.
      mask init:
      | xps_xsg_conf_mask;
      mask Help: eval('xlWeb([getenv(''MLIB_ROOT''), ''\doc\html\sys_xsg_core_config\sys_xsg_core_config.html''])')
      mask TypeOptions hw_sys: ROACH:sx95t | ROACH:lx110t | ROACH2:sx475t | SNAP:xc7k160t | KC705:xc7k325t | SKARAB:xc7vx690t
      mask Callback hw_sys: xps_xsg_conf_callback
      mask TypeOptions clk_src: sys_clk | aux_clk
      mask Callback clk_src: xps_xsg_conf_callback
      mask Callback clk_rate: xps_xsg_conf_callback
      mask TypeOptions synthesis_tool: Leonardo Spectrum | Synplify | Synplify Pro | XST
      mask Display: fprintf(['MSSGE\n', hw_sys]);
  tag scope: cnt_rst=global, ct_chans_per_x=global, ct_fake_data_error=global, ct_num_xeng=global, ct_num_xeng_recip=global, ct_rst_err_latch=global, ct_tag_insert_sel=global, ct_tvg_en2=global, ct_tvg_en=global, flag_pktfreq=global, flag_pktfreq_g=global, flag_pktstart=global, pfb_bypass=global, pktoffset_sel=global, pktstart_sel=global, sys_rst=global, ts_tvg_en=global, tvgtone_levels=global, tvgtone_p0=global, tvgtone_p1=global, up_timestep_error=global
  wires:
  Constant3/1 -> gbe0/8(rx_overrun_ack)
  Constant4/1 -> gbe0/7(rx_ack)
  [gbe_rst] -> pipeline99/1(d)
  unpack_and_reorder/5(recvd) -> ts_tvg/6(recvd_in)
  sync_gen/2(dout) -> bus_expand6/1(bus_in)
  sync_gen/3(dvalid) -> impulse_gen0/6(en), impulse_gen1/6(en)
  Slice4/1 -> pipeline16/1(d)
  pipeline16/1(q) -> local_time_lsw/1(out_timestamp_lsw)
  Slice16/1 -> Convert6/1
  pipeline47/1(q) -> local_time_msw/1(out_timestamp_msw)
  Convert6/1 -> pipeline47/1(d)
  [time80_48] -> Slice16/1, Slice4/1
  bus_expand17/1(msb_out2) -> [unpack_recvd0]
  bus_expand17/2(lsb_out1) -> [unpack_recvd1]
  Slice12/1 -> [time80]
  impulse_gen0/3(dvalid) -> [valid80]
  impulse_gen0/1(sync_out) -> [sync80]
  impulse_gen0/2(dout) -> [d80_adc0]
  impulse_gen0/4(misco) -> [time80_48], Slice12/1
  [tvg_adc0_en] -> impulse_gen0/1(tvg_en)
  impulse_gen1/1(sync_out) -> Terminator6/1
  impulse_gen1/2(dout) -> [d80_adc1]
  impulse_gen1/3(dvalid) -> Terminator8/1
  impulse_gen1/4(misco) -> [dig_flags]
  [tvg_adc1_en] -> impulse_gen1/1(tvg_en)
  impulse0/1(in_offset) -> Slice7/1
  impulse0/2(in_amplitude) -> impulse_gen0/3(impulse_amplitude)
  impulse1/1(in_offset) -> Slice8/1
  impulse1/2(in_amplitude) -> impulse_gen1/3(impulse_amplitude)
  sync_gen/1(sync) -> impulse_gen0/4(sync_in), impulse_gen1/4(sync_in)
  bus_expand6/1(msb_out2) -> impulse_gen0/5(din)
  bus_expand6/2(lsb_out1) -> impulse_gen1/5(din)
  sync_gen/5(misco) -> impulse_gen1/7(misci)
  sync_gen/4(time_out) -> impulse_gen0/7(misci)
  Constant31/1 -> Concat9/2
  [unpack_timestamp] -> Concat9/1
  [up_timestep_error] -> Logical15/1
  [sys_rst] -> Logical15/2
  Logical15/1 -> edge_detect17/1(in)
  edge_detect17/1(out) -> [sys_relock]
  Concat9/1 -> sync_gen/1(time_in)
  [sys_relock] -> sync_gen/5(relock)
  [unpack_dv] -> sync_gen/2(en)
  [unpack_d160] -> sync_gen/3(din)
  Slice7/1 -> impulse_gen0/2(impulse_offset)
  Slice8/1 -> impulse_gen1/2(impulse_offset)
  trig_time_msw/1(in_msw) -> pipeline28/1(d)
  trig_time_lsw/1(in_lsw) -> pipeline44/1(d)
  Concat13/1 -> Relational10/1
  pipeline28/1(q) -> Concat13/1
  pipeline44/1(q) -> Concat13/2
  [valid80] -> Counter/2
  [sync80] -> Counter/1
  Constant12/1 -> Relational7/2
  Counter/1 -> Relational7/1
  Relational10/1 -> Mux/2
  Relational7/1 -> Mux/3
  [valid80] -> Delay49/1
  Logical12/1 -> Logical14/1
  Logical14/1 -> [adc_snap_trig]
  [adc_snap_arm] -> Logical14/2
  [time80_48] -> Relational10/2
  Delay49/1 -> Logical12/2
  Mux/1 -> Logical12/1
  [adc_snap_trig_source] -> Mux/1
  iptx_base/1(in_reg) -> pipeline105/1(d)
  pipeline105/1(q) -> [tx_ip_base]
  tx_metadata/1(in_porttx) -> pipeline106/1(d)
  tx_metadata/2(in_board_id) -> pipeline107/1(d)
  pipeline106/1(q) -> [tx_port]
  pipeline107/1(q) -> [tx_board_id]
  edge_detect4/1(out) -> pipeline5/1(d)
  control/7(in_cnt_rst) -> edge_detect1/1(in)
  edge_detect1/1(out) -> pipeline14/1(d)
  control/3(in_gbe_rst) -> pipeline6/1(d)
  control/1(in_sys_rst) -> pipeline3/1(d)
  pipeline3/1(q) -> [sys_rst]
  pipeline5/1(q) -> [clr_status]
  pipeline6/1(q) -> [gbe_rst]
  pipeline7/1(q) -> [gbe_txen]
  pipeline13/1(q) -> [tvg_adc0_en]
  pipeline14/1(q) -> [cnt_rst]
  control/5(in_tvg_adc0) -> pipeline13/1(d)
  edge_detect2/1(out) -> pipeline38/1(d)
  pipeline38/1(q) -> [gbe_cnt_rst]
  control/8(in_gbe_cnt_rst) -> edge_detect2/1(in)
  control/4(in_gbe_txen) -> pipeline7/1(d)
  control/2(in_status_clr) -> edge_detect4/1(in)
  pipeline43/1(q) -> [adc_snap_arm]
  control/9(in_adc_snap_arm) -> pipeline43/1(d)
  control/10(in_adc_snap_trig_select) -> pipeline39/1(d)
  pipeline39/1(q) -> [adc_snap_trig_source]
  pfb/2(dout0) -> [pfb_d144_0]
  pfb/3(dout1) -> [pfb_d144_1]
  fft_shift/1(in_fft_shift) -> pipeline4/1(d)
  pfb/5(of) -> [pfb_of]
  pfb/4(dvalid) -> [pfb_dv]
  pfb/1(sync_out) -> [pfb_sync]
  [pfbin_d1] -> pfb/3(din1)
  [pfbin_d0] -> pfb/2(din0)
  [pfbin_sync] -> pfb/1(sync_in)
  [pfbin_dv] -> pfb/4(en)
  tl_fd0/2(enable) -> phase_compensation0/5(load_value)
  tl_fd1/1(value) -> phase_compensation1/4(delay_value)
  tl_fd1/2(enable) -> phase_compensation1/5(load_value)
  tl_fd0/1(value) -> phase_compensation0/4(delay_value)
  [clr_status] -> tl_fd1/1(rst), tl_fd0/1(rst)
  phase_compensation0/1(sync_out) -> [fdfs_sync]
  phase_compensation1/1(sync_out) -> Terminator24/1
  phase_compensation0/2(dout) -> [fdfs_d144_0]
  phase_compensation1/2(dout) -> [fdfs_d144_1]
  phase_compensation0/3(dvalid) -> [fdfs_dv]
  phase_compensation1/3(dvalid) -> Terminator25/1
  [ld_val0] -> tl_fd0/3(load_value)
  [ld_val1] -> tl_fd1/3(load_value)
  bus_expand16/1(msb_out2) -> tl_fd0/5(din)
  tl_fd0/5(dvalid) -> phase_compensation0/3(en)
  tl_fd0/3(sync_out) -> phase_compensation0/1(sync_in)
  tl_fd0/4(dout) -> phase_compensation0/2(din)
  tl_fd1/4(dout) -> phase_compensation1/2(din)
  bus_expand16/2(lsb_out1) -> tl_fd1/5(din)
  Constant29/1 -> Concat2/2
  Concat2/1 -> tl_fd1/2(current_time), tl_fd0/2(current_time)
  [gbe_cnt_rst] -> pipeline31/1(d)
  pipeline31/1(q) -> gbe0/9(debug_rst)
  Counter2/1 -> pipeline29/1(d)
  Constant26/1 -> eq1/2(data_in)
  Constant11/1 -> eq1/3(we)
  Delay53/1 -> quant1/1(sync_in)
  Delay34/1 -> quant1/2(din)
  eq1/1(data_out) -> quant1/4(coeffs)
  Delay50/1 -> quant1/3(en)
  Counter4/1 -> pipeline27/1(d)
  Constant24/1 -> eq0/2(data_in)
  Constant25/1 -> eq0/3(we)
  Delay51/1 -> quant0/1(sync_in)
  Delay2/1 -> quant0/2(din)
  Delay52/1 -> quant0/3(en)
  eq0/1(data_out) -> quant0/4(coeffs)
  quant0/1(sync_out) -> [q_sync]
  quant0/2(dout) -> [q_d64_0]
  quant0/3(dvalid) -> [q_dv]
  quant0/4(of) -> [q_of0]
  quant1/2(dout) -> [q_d64_1]
  quant1/1(sync_out) -> Terminator19/1
  quant1/3(dvalid) -> Terminator21/1
  quant1/4(of) -> [q_of1]
  pipeline27/1(q) -> eq0/1(addr)
  pipeline29/1(q) -> eq1/1(addr)
  [q_sync] -> generate_pkt_sync0/1(sync)
  Concat/1 -> generate_pkt_sync0/3(data)
  generate_pkt_sync0/1(out_sync) -> Terminator18/1
  [q_d64_0] -> Concat/1
  [q_d64_1] -> Concat/2
  bus_expand14/1(msb_out2) -> bus_expand12/1(bus_in)
  bus_expand14/2(lsb_out1) -> bus_expand13/1(bus_in)
  [q_dv] -> generate_pkt_sync0/2(valid)
  [fdfs_sync] -> Delay51/1, pipeline42/1(d)
  [fdfs_d144_0] -> Delay2/1
  [fdfs_dv] -> Delay52/1, pipeline41/1(d)
  pipeline41/1(q) -> Counter4/2
  pipeline42/1(q) -> Counter4/1
  pipeline45/1(q) -> Counter2/2
  [fdfs_sync] -> Delay53/1, pipeline48/1(d)
  [fdfs_d144_1] -> Delay34/1
  [fdfs_dv] -> Delay50/1, pipeline45/1(d)
  pipeline48/1(q) -> Counter2/1
  generate_pkt_sync0/3(out_data) -> pipeline30/1(d)
  generate_pkt_sync0/2(out_valid) -> pipeline32/1(d), pipeline49/1(d)
  generate_pkt_sync0/4(packet_sync) -> pipeline46/1(d), pipeline50/1(d)
  pipeline30/1(q) -> bus_expand14/1(bus_in)
  pipeline32/1(q) -> snap_quant0/9(we)
  pipeline46/1(q) -> snap_quant0/10(trig)
  pipeline49/1(q) -> snap_quant1/9(we)
  pipeline50/1(q) -> snap_quant1/10(trig)
  gbe0/13(rx_dest_ip) -> pipeline115/1(d)
  gbe0/14(rx_dest_port) -> pipeline116/1(d)
  [rx_dest_ip] -> pipeline/1(d)
  pipeline/1(q) -> rx_dest_ip/1(out_reg)
  [rx_dest_port] -> pipeline18/1(d)
  pipeline18/1(q) -> rx_dest_port/1(out_reg)
  gbe0/1(led_up) -> pipeline100/1(d)
  [forty_gbe_led_up] -> pipeline19/1(d)
  gbe0/2(led_rx) -> pipeline101/1(d)
  [forty_gbe_led_rx] -> pipeline20/1(d)
  gbe0/3(led_tx) -> pipeline102/1(d)
  [forty_gbe_led_tx] -> pipeline51/1(d)
  gbe0/4(tx_afull) -> pipeline103/1(d)
  gbe0/5(tx_overflow) -> pipeline104/1(d)
  gbe0/12(rx_overrun) -> pipeline114/1(d)
  pipeline19/1(q) -> gbe_status/1(out_led_up)
  pipeline20/1(q) -> gbe_status/2(out_led_rx)
  pipeline51/1(q) -> gbe_status/3(out_led_tx)
  gbe0/8(rx_source_ip) -> pipeline110/1(d)
  gbe0/9(rx_source_port) -> pipeline111/1(d)
  pipeline55/1(q) -> rx_src_ip/1(out_reg)
  pipeline56/1(q) -> rx_src_port/1(out_reg)
  [forty_gbe_rx_src_port] -> pipeline56/1(d)
  [forty_gbe_rx_src_ip] -> pipeline55/1(d)
  gbe0/6(rx_data) -> pipeline108/1(d)
  gbe0/10(rx_end_of_frame) -> pipeline112/1(d)
  gbe0/11(rx_bad_frame) -> pipeline113/1(d)
  pipeline80/1(q) -> [flag_sync]
  pipeline81/1(q) -> [flag_misc]
  pipeline82/1(q) -> [flag_dvalid]
  pipeline83/1(q) -> [flag_time]
  pipeline85/1(q) -> time_gen1/4(rd_sync_in)
  pipeline87/1(q) -> time_gen1/6(rd_misc_in)
  [s256_d] -> pipeline98/1(d)
  [s256_ip] -> pipeline97/1(d)
  [s256_port] -> pipeline96/1(d)
  Logical2/1 -> gbe0/6(tx_end_of_frame)
  [s256_v] -> Logical1/2
  [s256_eof] -> Logical2/2
  Delay1/1 -> Logical1/1, Logical2/1
  [s256_eof] -> Delay1/2
  pipeline96/1(q) -> gbe0/5(tx_dest_port)
  pipeline97/1(q) -> gbe0/4(tx_dest_ip)
  pipeline98/1(q) -> gbe0/2(tx_data)
  pipeline99/1(q) -> gbe0/1(rst)
  [gbe_txen] -> Delay1/1
  pipeline100/1(q) -> [forty_gbe_led_up]
  pipeline101/1(q) -> [forty_gbe_led_rx]
  pipeline102/1(q) -> [forty_gbe_led_tx]
  pipeline103/1(q) -> [forty_gbe_tx_full]
  pipeline104/1(q) -> [forty_gbe_tx_of]
  pipeline108/1(q) -> [forty_gbe_rx_data]
  pipeline110/1(q) -> [forty_gbe_rx_src_ip]
  pipeline111/1(q) -> [forty_gbe_rx_src_port]
  pipeline112/1(q) -> [forty_gbe_rx_eof]
  pipeline113/1(q) -> [forty_gbe_rx_bad]
  pipeline114/1(q) -> [forty_gbe_rx_overrun]
  pipeline115/1(q) -> [rx_dest_ip]
  pipeline116/1(q) -> [rx_dest_port]
  [forty_gbe_rx_data] -> unpack_and_reorder/1(d256)
  [forty_gbe_rx_valid] -> unpack_and_reorder/2(dv256)
  [forty_gbe_rx_eof] -> unpack_and_reorder/3(eof256)
  unpack_and_reorder/2(d160) -> ts_tvg/3(data_in)
  unpack_and_reorder/3(dv) -> ts_tvg/4(dv_in)
  unpack_and_reorder/4(time) -> ts_tvg/5(time_in)
  unpack_and_reorder/1(sync) -> ts_tvg/2(sync_in)
  Inverter1/1 -> Logical6/1
  [unpack_recvd0] -> Inverter1/1
  [unpack_dv] -> Logical6/2
  Inverter2/1 -> Logical7/1
  [unpack_recvd1] -> Inverter2/1
  [unpack_dv] -> Logical7/2
  Logical7/1 -> Logical/2
  Logical6/1 -> Logical/1
  Logical/1 -> [unpack_missing]
  pipeline10/1(q) -> [unpack_sync]
  pipeline11/1(q) -> [unpack_d160]
  pipeline12/1(q) -> [unpack_dv]
  pipeline15/1(q) -> [unpack_timestamp]
  pipeline17/1(q) -> bus_expand17/1(bus_in)
  [clr_status] -> Subsystem5/1(rst)
  [up_dbg_rst] -> Subsystem4/1(rst)
  [upg_sp_dv] -> Logical3/2
  [upg_sp_eof] -> Logical3/1
  [upg_sperr_magic] -> Subsystem4/2(in0)
  [upg_sperr_len] -> Subsystem4/5(in3)
  [upg_sperr_hdr] -> Subsystem4/3(in1)
  [upg_sperr_pad] -> Subsystem4/4(in2)
  Delay/1 -> pipeline85/1(d)  "gapsync"
  Delay3/1 -> pipeline86/1(d)  "gapdata"
  Mux1/1 -> pipeline87/1(d)  "gapvalid"
  tl_fd0/7(misco) -> Terminator2/1
  tl_fd0/6(time) -> Terminator3/1
  tl_fd1/6(time) -> Terminator4/1
  tl_fd1/3(sync_out) -> phase_compensation1/1(sync_in)
  tl_fd1/5(dvalid) -> phase_compensation1/3(en)
  tl_fd1/7(misco) -> Terminator5/1
  Constant18/1 -> tl_fd0/7(misci)
  Constant19/1 -> tl_fd1/7(misci)
  Subsystem4/5(out4) -> spead_status/5(out_pkt_cnt)
  Logical3/1 -> Subsystem4/6(in4)
  Constant1/1 -> sync_gen/4(misci)
  time_gen/1(rd_sync_out) -> tl_fd1/4(sync_in), tl_fd0/4(sync_in)
  time_gen/2(rd_dvalid) -> tl_fd1/6(en), tl_fd0/6(en)
  time_gen/3(rd_val_out) -> Concat2/1
  time_gen/4(rd_misc_out) -> bus_expand16/1(bus_in)
  [sync80] -> time_gen/1(wr_sync_in)
  [valid80] -> time_gen/2(wr_en)
  [pfb_sync] -> time_gen/4(rd_sync_in)
  [pfb_dv] -> time_gen/5(rd_en)
  [pfb_d144_1] -> Concat1/2
  [pfb_d144_0] -> Concat1/1
  Concat1/1 -> time_gen/6(rd_misc_in)
  [q_sync] -> time_gen1/1(wr_sync_in)
  [q_dv] -> time_gen1/2(wr_en)
  [time80] -> Slice2/1
  pipeline86/1(q) -> time_gen1/5(rd_en)
  time_gen1/1(rd_sync_out) -> pipeline80/1(d)
  time_gen1/4(rd_misc_out) -> pipeline81/1(d)
  time_gen1/2(rd_dvalid) -> pipeline82/1(d)
  time_gen1/3(rd_val_out) -> pipeline83/1(d)
  bus_expand12/1(msb_out8) -> snap_quant0/1(in_real0)
  bus_expand12/2(out7) -> snap_quant0/2(in_imag0)
  bus_expand12/3(out6) -> snap_quant0/3(in_real1)
  bus_expand12/4(out5) -> snap_quant0/4(in_imag1)
  bus_expand12/5(out4) -> snap_quant0/5(in_real2)
  bus_expand12/6(out3) -> snap_quant0/6(in_imag2)
  bus_expand12/7(out2) -> snap_quant0/7(in_real3)
  bus_expand12/8(lsb_out1) -> snap_quant0/8(in_imag3)
  bus_expand13/1(msb_out8) -> snap_quant1/1(in_real0)
  bus_expand13/2(out7) -> snap_quant1/2(in_imag0)
  bus_expand13/3(out6) -> snap_quant1/3(in_real1)
  bus_expand13/4(out5) -> snap_quant1/4(in_imag1)
  bus_expand13/5(out4) -> snap_quant1/5(in_real2)
  bus_expand13/6(out3) -> snap_quant1/6(in_imag2)
  bus_expand13/7(out2) -> snap_quant1/7(in_real3)
  bus_expand13/8(lsb_out1) -> snap_quant1/8(in_imag3)
  [time80] -> time_gen/3(wr_val_in)
  Slice2/1 -> time_gen1/3(wr_val_in)
  pipeline4/1(q) -> [fft_shift]
  Logical1/1 -> gbe0/3(tx_valid)
  pipeline59/1(q) -> [ct_tvg_en]
  control/11(in_ct_tvg_en) -> pipeline59/1(d)
  [delay_d0] -> Delay8/1
  bus_expand/1(msb_out8) -> snap_pre_pfb0/1(in_d0)
  bus_expand/3(out6) -> snap_pre_pfb0/3(in_d2)
  bus_expand/4(out5) -> snap_pre_pfb0/4(in_d3)
  bus_expand/6(out3) -> snap_pre_pfb0/6(in_d5)
  bus_expand/5(out4) -> snap_pre_pfb0/5(in_d4)
  bus_expand/7(out2) -> snap_pre_pfb0/7(in_d6)
  bus_expand/8(lsb_out1) -> snap_pre_pfb0/8(in_d7)
  bus_expand/2(out7) -> snap_pre_pfb0/2(in_d1)
  Constant8/1 -> Relational1/2
  Counter6/1 -> Relational1/1
  Relational1/1 -> snap_pre_pfb0/10(trig)
  Delay8/1 -> bus_expand/1(bus_in)
  Delay9/1 -> snap_pre_pfb0/9(we)
  [delay_d1] -> Delay10/1
  bus_expand4/1(msb_out8) -> snap_pre_pfb1/1(in_d0)
  bus_expand4/3(out6) -> snap_pre_pfb1/3(in_d2)
  bus_expand4/4(out5) -> snap_pre_pfb1/4(in_d3)
  bus_expand4/6(out3) -> snap_pre_pfb1/6(in_d5)
  bus_expand4/5(out4) -> snap_pre_pfb1/5(in_d4)
  bus_expand4/7(out2) -> snap_pre_pfb1/7(in_d6)
  bus_expand4/8(lsb_out1) -> snap_pre_pfb1/8(in_d7)
  bus_expand4/2(out7) -> snap_pre_pfb1/2(in_d1)
  [delay_dv] -> Delay11/1, Counter7/2
  [delay_sync] -> Counter7/1
  Constant9/1 -> Relational2/2
  Counter7/1 -> Relational2/1
  Relational2/1 -> snap_pre_pfb1/10(trig)
  Delay10/1 -> bus_expand4/1(bus_in)
  Delay11/1 -> snap_pre_pfb1/9(we)
  pipeline52/1(q) -> [up_dbg_rst]
  control/12(in_unpack_debug_reset) -> pipeline52/1(d)
  Subsystem4/4(out3) -> spead_status/4(out_pkt_len_err_cnt)
  Subsystem4/3(out2) -> spead_status/3(out_pad_err_cnt)
  Subsystem4/2(out1) -> spead_status/2(out_header_err_cnt)
  Subsystem4/1(out0) -> spead_status/1(out_magic_err_cnt)
  [clr_status] -> Subsystem3/1(rst)
  Slice/1 -> Subsystem3/2(in0)
  [pfb_of] -> Slice/1, Slice6/1
  Slice6/1 -> Subsystem3/3(in1)
  [pfb_sync] -> Subsystem3/4(in2)
  Subsystem3/3(out2) -> pfb_status/3(out_sync_cnt)
  Subsystem5/1(out0) -> quant_status/1(out_pol0_or_cnt)
  Relational/1 -> Subsystem5/2(in0)
  Constant10/1 -> Relational/2
  [q_of0] -> Relational/1
  Relational3/1 -> Subsystem5/3(in1)
  [q_of1] -> Relational3/1
  Constant13/1 -> Relational3/2
  Subsystem5/2(out1) -> quant_status/2(out_pol1_or_cnt)
  Subsystem3/1(out0) -> pfb_status/1(out_pol0_or_err_cnt)
  Subsystem3/2(out1) -> pfb_status/2(out_pol1_or_err_cnt)
  [delay_dv] -> Counter6/2, Delay9/1
  [delay_sync] -> Counter6/1
  [q_sync] -> hmc_ct/1(in_sync)
  [q_d64_1] -> Concat4/1
  [q_dv] -> hmc_ct/2(in_dv)
  [q_d64_0] -> Concat4/2
  Concat4/1 -> [q_d128], hmc_ct/3(in_d128)
  [ct_tvg_en2] -> Mux1/1
  [ct_dvalid] -> Delay5/1
  Delay6/1 -> Mux1/2
  Delay7/1 -> tvg/1(sync), Delay/1
  [ct_s] -> Delay7/1
  [ct_data] -> Delay6/1
  Delay5/1 -> tvg/2(dv), Delay3/1
  tvg/1(data256) -> Mux1/3
  pipeline129/1(q) -> pipeline142/1(d)
  pipeline141/1(q) -> pipeline129/1(d)
  [q_dv] -> qt_block_check/1(dv)
  [cnt_rst] -> Subsystem12/1(rst)
  Subsystem12/1(out0) -> qt_dv_err/1(out_dvblock_err_cnt)
  qt_block_check/1(error) -> Subsystem12/2(in0)
  [cd_bypass] -> Mux4/1
  [cd_bypass] -> Mux2/1
  Mux4/1 -> [pfbin_sync]
  Mux2/1 -> [pfbin_dv]
  [cd_bypass] -> Mux3/1
  Mux3/1 -> [pfbin_d0]
  [cd_bypass] -> Mux5/1
  Mux5/1 -> [pfbin_d1]
  control/13(in_cd_bypass) -> pipeline131/1(d)
  pipeline131/1(q) -> [cd_bypass]
  Concat22/1 -> [ld_val0]
  Concat3/1 -> [ld_val1]
  phase0/1(in_initial) -> Reinterpret2/1
  delta_delay0/1(in_delta) -> Reinterpret1/1
  phase0/2(in_delta) -> Reinterpret3/1
  Reinterpret8/1 -> Concat22/1
  Reinterpret1/1 -> Concat22/2
  Reinterpret2/1 -> Concat22/3
  Reinterpret3/1 -> Concat22/4
  phase1/1(in_initial) -> Reinterpret5/1
  delta_delay1/1(in_delta) -> Reinterpret4/1
  phase1/2(in_delta) -> Reinterpret6/1
  Reinterpret4/1 -> Concat3/2
  Reinterpret5/1 -> Concat3/3
  Reinterpret6/1 -> Concat3/4
  Reinterpret7/1 -> Concat3/1
  delay0/1(in_initial) -> Reinterpret8/1
  delay1/1(in_initial) -> Reinterpret7/1
  [clr_status] -> Subsystem2/1(rst)
  [cd_error_p0] -> Subsystem2/2(in0)
  [ct_dv] -> Subsystem8/1(In1)
  Subsystem8/1(Out1) -> ct_dv_rate/1(out_reg)
  Constant14/1 -> ct_control1/1(sim_1)
  Constant5/1 -> ct_control1/2(sim_2)
  Constant7/1 -> ct_control1/3(sim_3)
  we_delay37/1(q) -> [ct_num_xeng]
  we_delay38/1(q) -> [ct_num_xeng_recip]
  we_delay39/1(q) -> [ct_chans_per_x]
  ct_control1/2(in_num_x_recip) -> we_delay38/1(d)
  ct_control1/3(in_chans_per_x) -> we_delay39/1(d)
  ct_control1/1(in_num_x) -> we_delay37/1(d)
  we_delay49/1(q) -> [ct_tag_insert_sel]
  edge_detect3/1 -> [ct_rst_err_latch]
  we_delay47/1(q) -> edge_detect3/1
  we_delay48/1(q) -> [ct_fake_data_error]
  we_delay13/1(q) -> [ct_tvg_en]
  we_delay50/1(q) -> [ct_tvg_en2]
  Constant2/1 -> ct_control0/5(sim_5)
  Constant21/1 -> ct_control0/4(sim_4)
  Constant20/1 -> ct_control0/3(sim_3)
  Constant22/1 -> ct_control0/2(sim_2)
  Constant15/1 -> ct_control0/1(sim_1)
  ct_control0/1(in_tvg_en) -> we_delay13/1(d)
  ct_control0/2(in_tvg_en2) -> we_delay50/1(d)
  ct_control0/3(in_rst_err_latch) -> we_delay47/1(d)
  ct_control0/4(in_fake_error) -> we_delay48/1(d)
  ct_control0/5(in_tag_insert) -> we_delay49/1(d)
  [cnt_rst] -> Subsystem10/1(rst)
  [obuf_ct_addr_err_g] -> Subsystem10/2(in0)
  [obuf_ct_addr_err2_g] -> Subsystem10/3(in1)
  Subsystem10/1(out0) -> ct_status1/1(out_addr_err0_cnt)
  Subsystem10/2(out1) -> ct_status1/2(out_addr_err1_cnt)
  Subsystem10/3(out2) -> ct_status1/3(out_sync_cnt)
  [ct_sync] -> Subsystem10/4(in2)
  [ct_pktstart] -> we_delay1/1(d)
  [ct_dv] -> we_delay2/1(d)
  we_delay1/1(q) -> pktlen_check/1(pkt_start)
  we_delay2/1(q) -> dv_block_check/1(dv), pktlen_check/2(dv)
  pktlen_check/1(error) -> we_delay7/1(d)
  dv_block_check/1(error) -> we_delay29/1(d)
  [cnt_rst] -> Subsystem6/1(rst)
  we_delay7/1(q) -> [ct_pktlen_err], Subsystem6/2(in0)
  we_delay29/1(q) -> [ct_dvblk_err], Subsystem6/3(in1)
  Subsystem6/1(out0) -> ct_dv_err/1(out_pktlen_err_cnt)
  Subsystem6/2(out1) -> ct_dv_err/2(out_dvblock_err_cnt)
  [cnt_rst] -> Subsystem9/1(rst)
  we_delay45/1(q) -> ct_status0/1(out_post)
  we_delay46/1(q) -> ct_status0/2(out_init)
  [hmc_postokay_g] -> we_delay45/1(d)
  [hmc_init_done_g] -> we_delay46/1(d)
  [hmc_wr_dv_g] -> Subsystem9/6(in4)
  [ct_bank_error_g] -> Subsystem9/2(in0)
  [hmc_err_wrrdy_g] -> Subsystem9/4(in2)
  [ct_en_sync_error_g] -> Subsystem9/3(in1)
  [hmc_err_rdrdy_g] -> Subsystem9/5(in3)
  Subsystem9/1(out0) -> ct_status0/3(out_err_bank)
  Subsystem9/3(out2) -> ct_status0/5(out_err_rdrdy)
  Subsystem9/2(out1) -> ct_status0/4(out_err_en_sync)
  Subsystem9/5(out4) -> ct_status0/7(out_wr_ctr)
  Subsystem9/4(out3) -> ct_status0/6(out_err_wrrdy)
  pipeline2/1(q) -> gbe_in_msb/1(in_d_msb)
  pipeline122/1(q) -> gbe_in_lsb/1(in_d_lsb)
  [s256_d] -> Slice3/1, Slice1/1
  Slice1/1 -> pipeline2/1(d)
  Slice3/1 -> pipeline122/1(d)
  [pack_snap_arm] -> Logical9/1, Logical8/1
  [s256_v] -> Logical8/2
  [s256_eof] -> Logical9/2
  Logical8/1 -> gbe_in_msb/2(we), gbe_in_lsb/2(we)
  Logical9/1 -> gbe_in_msb/3(trig), gbe_in_lsb/3(trig)
  [ct_snap_err_stop] -> pipeline8/1(d)
  pipeline8/1(q) -> gbe_in_msb/4(stop), gbe_in_lsb/4(stop)
  [gbe_stopmux] -> multimux4/1(select)
  [forty_gbe_tx_of] -> multimux4/2(input1)
  [forty_gbe_tx_full] -> multimux4/3(input2)
  [forty_gbe_tx_err] -> multimux4/4(input3)
  [pack_dv_err] -> multimux4/5(input4)
  [flag_dvalid] -> Subsystem13/1(In1)
  Subsystem13/1(Out1) -> time_status/1(out_dv_cnt)
  hmc_ct/4(pkt_start) -> [ct_pktstart], Delay33/1
  hmc_ct/1(out_sync) -> [ct_sync]
  hmc_ct/2(out_dv) -> [ct_dv]
  hmc_ct/3(out_d256) -> [ct_d256]
  hmc_ct/5(freq_id) -> [ct_pktfreq], Delay35/1
  pipeline139/1(q) -> pipeline140/1(d)
  pipeline140/1(q) -> pipeline141/1(d)
  pipeline142/1(q) -> [flag_pktstart]
  [s256_v] -> Subsystem11/1(In1)
  Subsystem11/1(Out1) -> pack_status/1(out_dv_cnt)
  pipeline121/1(q) -> Convert/1
  pipeline124/1(q) -> [ip_per_x]
  pipeline125/1(q) -> [num_x]
  x_setup/1(in_f_per_x) -> pipeline121/1(d)
  x_setup/2(in_ip_per_x) -> pipeline124/1(d)
  x_setup/3(in_num_x) -> pipeline125/1(d)
  pipeline120/1(q) -> [pack_snap_arm]
  x_setup/4(in_snap_arm) -> pipeline120/1(d)
  pipeline130/1(q) -> [pktstart_sel]
  x_setup/5(in_pktstart_mux) -> pipeline130/1(d)
  [s256_v] -> pack_block_check/1(dv)
  [cnt_rst] -> Subsystem14/1(rst)
  Subsystem14/1(out0) -> pack_dv_err/1(out_dvblock_err_cnt)
  pack_block_check/1(error) -> [pack_dv_err], Subsystem14/2(in0)
  pipeline149/1(q) -> [pack_mux]
  x_setup/6(in_pack_mux) -> pipeline149/1(d)
  pipeline151/1(q) -> pipeline152/1(d)
  pipeline152/1(q) -> pipeline153/1(d)
  pipeline153/1(q) -> pipeline154/1(d)
  pipeline154/1(q) -> pipeline155/1(d)
  pipeline155/1(q) -> [flag_pktfreq]
  [flag_pktfreq] -> [flag_pktfreq_g], pipeline159/1(d)
  pipeline158/1(q) -> [s256_pktfreq]
  pipeline159/1(q) -> pipeline158/1(d)
  [q_sync] -> Register3/3, Register3/1
  Register3/1 -> Register7/1
  [q_dv] -> Register7/2
  Register7/1 -> edge_detect7/1
  edge_detect7/1 -> Register3/2, Register1/2, Register8/2
  [time80_48] -> Slice40/1, Slice35/1
  Slice35/1 -> Delay15/1
  Delay15/1 -> Register8/1
  Register8/1 -> ct_sync_time_msw/1(out_reg)
  Register1/1 -> ct_sync_time_lsw/1(out_reg)
  Slice40/1 -> Delay19/1
  Delay19/1 -> Register1/1
  [flag_sync] -> Register5/3, Register5/1
  Register5/1 -> Register6/1
  [flag_dvalid] -> Register6/2
  Register6/1 -> edge_detect6/1
  edge_detect6/1 -> Register4/2, Register9/2, Register5/2
  [pack_sync_time] -> Slice41/1, Slice36/1
  Slice36/1 -> Delay14/1
  Delay14/1 -> Register9/1
  Register9/1 -> pack_sync_time_msw/1(out_reg)
  Register4/1 -> pack_sync_time_lsw/1(out_reg)
  Slice41/1 -> Delay20/1
  Delay20/1 -> Register4/1
  multimux4/1(output) -> [ct_snap_err_stop]
  [cnt_rst] -> Subsystem16/1(rst)
  [freq_sync_error] -> Subsystem16/3(in1)
  [rd_go_err_g] -> Subsystem16/2(in0)
  Subsystem16/1(out0) -> ct_status2/1(out_out_go_err)
  Subsystem16/2(out1) -> ct_status2/2(out_freq_sync_err)
  [ct_d256] -> Slice43/1
  Slice43/1 -> Relational21/2
  [ct_pktfreq] -> Relational21/1
  Relational21/1 -> Logical16/2
  [ct_dv] -> Delay4/1
  Delay4/1 -> Logical16/1
  Logical16/1 -> [freq_sync_error]
  tl_cd0_control0/3(in_load_time_msw) -> Concat6/1
  tl_cd0_control/1(in_load_time_lsw) -> Concat6/2
  Constant42/1 -> tl_cd0_control/1(sim_1)
  Constant40/1 -> tl_cd0_control0/3(sim_3)
  Constant41/1 -> tl_cd0_control0/2(sim_2)
  Constant43/1 -> Delay12/1
  Delay12/1 -> tl_cd0_control0/1(sim_1)
  Concat6/1 -> pipeline136/1(d)
  tl_cd0_control0/2(in_load_immediate) -> pipeline135/1(d)
  tl_cd0_control0/1(in_arm) -> pipeline134/1(d)
  tl_cd1_control0/3(in_load_time_msw) -> Concat8/1
  tl_cd1_control/1(in_load_time_lsw) -> Concat8/2
  Constant47/1 -> tl_cd1_control/1(sim_1)
  Constant45/1 -> tl_cd1_control0/3(sim_3)
  Constant46/1 -> tl_cd1_control0/2(sim_2)
  Constant48/1 -> Delay13/1
  Delay13/1 -> tl_cd1_control0/1(sim_1)
  Concat8/1 -> pipeline143/1(d)
  tl_cd1_control0/2(in_load_immediate) -> pipeline138/1(d)
  tl_cd1_control0/1(in_arm) -> pipeline137/1(d)
  [ld_val0] -> pipeline73/1(d)
  [clr_status] -> pipeline25/1(d), pipeline75/1(d)
  tl_cd0/6(time) -> [time80_tl_cd0]
  Constant6/1 -> Concat15/2
  Concat15/1 -> pipeline24/1(d), Gateway Out7/1, pipeline74/1(d)
  [time80] -> Concat15/1
  pipeline75/1(q) -> tl_cd0/1(rst)
  pipeline74/1(q) -> tl_cd0/2(current_time)
  pipeline73/1(q) -> tl_cd0/3(load_value)
  pipeline72/1(q) -> tl_cd0/4(sync_in)
  pipeline71/1(q) -> tl_cd0/5(din)
  pipeline76/1(q) -> tl_cd0/6(en)
  [sync80] -> pipeline36/1(d), pipeline72/1(d)
  [valid80] -> pipeline34/1(d), pipeline76/1(d)
  Constant16/1 -> tl_cd0/7(misci)
  tl_cd0/7(misco) -> Terminator/1
  tl_cd0/3(sync_out) -> [sync_tl_cd0]
  tl_cd0/5(dvalid) -> [dvalid_tl_cd0]
  tl_cd0/4(dout) -> [dout_tl_cd0]
  tl_cd0/2(enable) -> [en_tl_cd0]
  tl_cd0/1(value) -> [delay_tl_cd0]
  pipeline92/1(q) -> tl_cd0/10(load_time)
  pipeline91/1(q) -> tl_cd0/9(load_immediate)
  pipeline90/1(q) -> tl_cd0/8(arm)
  [tl_cd0_arm] -> pipeline90/1(d)
  [tl_cd0_load_immediate] -> pipeline91/1(d)
  [tl_cd0_load_time] -> pipeline92/1(d)
  Gateway Out7/1 -> To Workspace7/1
  [d80_adc0] -> pipeline71/1(d)
  cd_compensation0/2(dout) -> [hmc_data_p0]
  cd_compensation0/4(hmc_error) -> [cd_error_p0]
  [dvalid_tl_cd0] -> Delay22/1
  [sync_tl_cd0] -> Delay21/1
  [en_tl_cd0] -> Delay24/1
  [delay_tl_cd0] -> Delay23/1
  Concat5/1 -> time_gen_cd/6(rd_misc_in)
  time_gen_cd/4(rd_misc_out) -> bus_expand2/1(bus_in)
  [sync_tl_cd0] -> time_gen_cd/1(wr_sync_in)
  [dvalid_tl_cd0] -> time_gen_cd/2(wr_en)
  [hmc_sync_p0] -> time_gen_cd/4(rd_sync_in)
  [hmc_dvalid_p0] -> time_gen_cd/5(rd_en)
  time_gen_cd/1(rd_sync_out) -> [tg_rd_sync]
  time_gen_cd/2(rd_dvalid) -> [tg_rd_dvalid]
  [dvalid_tl_bs0] -> wb_prog_delay/4(en)
  [delay_tl_bs0] -> wb_prog_delay/2(delay_val)
  [delay_tl_sync0] -> wb_prog_delay/1(sync)
  [en_tl_bs0] -> wb_prog_delay/5(load_val)
  wb_prog_delay/2(data_out) -> [delay_d0]
  wb_prog_delay/3(dvalid) -> [delay_dv]
  [time80_tl_cd0] -> Slice9/1
  Slice9/1 -> time_gen_cd/3(wr_val_in)
  Constant35/1 -> Concat7/2
  time_gen_cd/3(rd_val_out) -> Concat7/1
  Concat7/1 -> [tg_rd_time_out]
  cd_compensation0/3(dvalid) -> [hmc_dvalid_p0]
  cd_compensation0/1(sync_out) -> [hmc_sync_p0]
  wb_prog_delay/1(sync_out) -> [delay_sync]
  pipeline77/1(q) -> tl_cd_bs0/1(rst)
  pipeline1/1(q) -> tl_cd_bs0/2(current_time)
  pipeline78/1(q) -> tl_cd_bs0/3(load_value)
  pipeline84/1(q) -> tl_cd_bs0/4(sync_in)
  pipeline88/1(q) -> tl_cd_bs0/5(din)
  pipeline89/1(q) -> tl_cd_bs0/6(en)
  [clr_status] -> pipeline77/1(d)
  [tg_rd_time_out] -> pipeline1/1(d)
  [ld_val0] -> pipeline78/1(d)
  [tg_rd_sync] -> pipeline84/1(d)
  [tg_rd_dvalid] -> pipeline89/1(d)
  Constant34/1 -> tl_cd_bs0/7(misci)
  tl_cd_bs0/7(misco) -> Terminator12/1
  tl_cd_bs0/4(dout) -> [data_tl_bs0]
  tl_cd_bs0/6(time) -> Terminator13/1
  tl_cd_bs0/5(dvalid) -> [dvalid_tl_bs0]
  tl_cd_bs0/1(value) -> [delay_tl_bs0]
  tl_cd_bs0/3(sync_out) -> [delay_tl_sync0]
  tl_cd_bs0/2(enable) -> [en_tl_bs0]
  pipeline21/1(q) -> tl_cd_bs0/8(arm)
  pipeline22/1(q) -> tl_cd_bs0/9(load_immediate)
  pipeline23/1(q) -> tl_cd_bs0/10(load_time)
  [tl_cd0_arm] -> pipeline21/1(d)
  [tl_cd0_load_immediate] -> pipeline22/1(d)
  [tl_cd0_load_time] -> pipeline23/1(d)
  [data_tl_bs0] -> wb_prog_delay/3(din)
  [tg_data_p0] -> pipeline88/1(d)
  pipeline25/1(q) -> tl_cd1/1(rst)
  [ld_val1] -> pipeline26/1(d)
  pipeline24/1(q) -> tl_cd1/2(current_time)
  pipeline26/1(q) -> tl_cd1/3(load_value)
  pipeline36/1(q) -> tl_cd1/4(sync_in)
  pipeline33/1(q) -> tl_cd1/5(din)
  pipeline34/1(q) -> tl_cd1/6(en)
  pipeline37/1(q) -> tl_cd1/9(load_immediate)
  pipeline35/1(q) -> tl_cd1/8(arm)
  pipeline40/1(q) -> tl_cd1/10(load_time)
  [tl_cd1_arm] -> pipeline35/1(d)
  [tl_cd1_load_immediate] -> pipeline37/1(d)
  [tl_cd1_load_time] -> pipeline40/1(d)
  Constant17/1 -> tl_cd1/7(misci)
  tl_cd1/1(value) -> [delay_tl_cd1]
  tl_cd1/2(enable) -> [en_tl_cd1]
  tl_cd1/3(sync_out) -> [sync_tl_cd1]
  tl_cd1/4(dout) -> [dout_tl_cd1]
  tl_cd1/5(dvalid) -> [dvalid_tl_cd1]
  tl_cd1/6(time) -> [time80_tl_cd1]
  tl_cd1/7(misco) -> Terminator1/1
  [delay_tl_cd1] -> Delay27/1
  [en_tl_cd1] -> Delay28/1
  [sync_tl_cd1] -> Delay25/1
  [dvalid_tl_cd1] -> Delay26/1
  cd_compensation1/1(sync_out) -> [hmc_sync_p1]
  cd_compensation1/2(dout) -> [hmc_data_p1]
  cd_compensation1/3(dvalid) -> [hmc_dvalid_p1]
  pipeline54/1(q) -> tl_cd_bs1/1(rst)
  pipeline53/1(q) -> tl_cd_bs1/2(current_time)
  pipeline60/1(q) -> tl_cd_bs1/3(load_value)
  pipeline61/1(q) -> tl_cd_bs1/4(sync_in)
  pipeline67/1(q) -> tl_cd_bs1/5(din)
  pipeline68/1(q) -> tl_cd_bs1/6(en)
  [clr_status] -> pipeline54/1(d)
  [tg_rd_time_out] -> pipeline53/1(d)
  [ld_val1] -> pipeline60/1(d)
  [tg_rd_sync] -> pipeline61/1(d)
  [tg_rd_dvalid] -> pipeline68/1(d)
  [tg_data_p1] -> pipeline67/1(d)
  Constant36/1 -> tl_cd_bs1/7(misci)
  pipeline156/1(q) -> tl_cd_bs1/8(arm)
  pipeline69/1(q) -> tl_cd_bs1/9(load_immediate)
  pipeline70/1(q) -> tl_cd_bs1/10(load_time)
  [tl_cd1_load_time] -> pipeline70/1(d)
  [tl_cd1_load_immediate] -> pipeline69/1(d)
  [tl_cd1_arm] -> pipeline156/1(d)
  tl_cd_bs1/7(misco) -> Terminator10/1
  tl_cd_bs1/4(dout) -> [data_tl_bs1]
  tl_cd_bs1/6(time) -> Terminator7/1
  tl_cd_bs1/5(dvalid) -> [dvalid_tl_bs1]
  tl_cd_bs1/1(value) -> [delay_tl_bs1]
  tl_cd_bs1/3(sync_out) -> [delay_tl_sync1]
  tl_cd_bs1/2(enable) -> [en_tl_bs1]
  [delay_tl_sync1] -> wb_prog_delay1/1(sync)
  [delay_tl_bs1] -> wb_prog_delay1/2(delay_val)
  [en_tl_bs1] -> wb_prog_delay1/5(load_val)
  [data_tl_bs1] -> wb_prog_delay1/3(din)
  [dvalid_tl_bs1] -> wb_prog_delay1/4(en)
  wb_prog_delay1/2(data_out) -> [delay_d1]
  wb_prog_delay1/1(sync_out) -> Terminator16/1
  wb_prog_delay1/3(dvalid) -> Terminator11/1
  [d80_adc1] -> pipeline33/1(d)
  tvg_tone_levels/2(in_p0i) -> bus_create/2(in2)
  tvg_tone_levels/3(in_p1r) -> bus_create/3(in3)
  tvg_tone_levels/4(in_p1i) -> bus_create/4(in4)
  tvg_tone_levels/1(in_p0r) -> bus_create/1(in1)
  tvg_tone_targets/1(in_p0) -> [tvgtone_p0]
  tvg_tone_targets/2(in_p1) -> [tvgtone_p1]
  Constant39/1 -> tvg_tone_targets/1(sim_1)
  Constant49/1 -> tvg_tone_targets/2(sim_2)
  Constant38/1 -> tvg_tone_levels/4(sim_4)
  Constant23/1 -> tvg_tone_levels/1(sim_1)
  Constant37/1 -> tvg_tone_levels/3(sim_3)
  Constant27/1 -> tvg_tone_levels/2(sim_2)
  bus_create/1(bus_out) -> [tvgtone_levels]
  Subsystem7/1(per_sec) -> reorder_status1/1(out_dv_per_sec)
  [upg_reo_time] -> Subsystem1/3(time)
  [upg_reo_recv] -> Subsystem1/4(recv)
  [upg_reo_dv] -> Subsystem7/1(dv), Subsystem1/2(dv)
  [up_dbg_rst] -> Subsystem1/1(rst)
  Subsystem1/7(time_change) -> [reo_time_change]
  Logical5/1 -> Subsystem1/7(overflow_err)
  [upg_of80_p1] -> Logical5/2
  [upg_of80_p0] -> Logical5/1
  Subsystem1/8(timestep_err) -> [up_timestep_error]
  [upg_reo_disc] -> Subsystem1/5(discard_err)
  [upg_reo_relock] -> Subsystem1/6(relock_err)
  Subsystem1/1(timestep_err_cnt) -> reorder_status/1(out_timestep_err_cnt)
  Subsystem1/2(recv_err_cnt) -> reorder_status/2(out_receive_err_cnt)
  Subsystem1/3(discard_err_cnt) -> reorder_status/3(out_discard_cnt)
  Subsystem1/4(relock_err_cnt) -> reorder_status/4(out_relock_err_cnt)
  Subsystem1/5(overflow_err_cnt) -> reorder_status/5(out_overflow_err_cnt)
  Subsystem1/6(dv_cnt) -> reorder_status/6(out_dv_cnt)
  pipeline93/1(q) -> [tvg_adc1_en]
  control/6(in_tvg_adc1) -> pipeline93/1(d)
  Constant/1 -> [forty_gbe_tx_err]
  pipeline57/1(q) -> bus_expand7/1(bus_in)
  pipeline163/1(q) -> bus_expand11/1(bus_in)
  [d80_adc1] -> pipeline163/1(d)
  [valid80] -> Slice5/1
  Slice14/1 -> pipeline162/1(d)
  [time80_48] -> Slice14/1
  pipeline162/1(q) -> snap_adc0/16(extra_timestamp)
  pipeline164/1(q) -> snap_adc1/5(we)
  Slice5/1 -> pipeline164/1(d), pipeline161/1(d)
  [d80_adc0] -> pipeline57/1(d)
  Delay43/1 -> snap_adc1/6(trig)
  pipeline160/1(q) -> bus_expand1/1(bus_in)
  [d80_adc1] -> pipeline160/1(d)
  [adc_snap_trig] -> snap_adc0/15(trig), Delay43/1
  bus_expand7/4(out5) -> snap_adc0/4(in_p0_d3)
  bus_expand7/5(out4) -> snap_adc0/5(in_p0_d4)
  bus_expand7/1(msb_out8) -> snap_adc0/1(in_p0_d0)
  bus_expand7/2(out7) -> snap_adc0/2(in_p0_d1)
  bus_expand7/3(out6) -> snap_adc0/3(in_p0_d2)
  bus_expand7/6(out3) -> snap_adc0/6(in_p0_d5)
  bus_expand7/7(out2) -> snap_adc0/7(in_p0_d6)
  bus_expand7/8(lsb_out1) -> snap_adc0/8(in_p0_d7)
  bus_expand1/1(msb_out6) -> snap_adc0/9(in_p1_d0)
  bus_expand1/2(out5) -> snap_adc0/10(in_p1_d1)
  bus_expand1/3(out4) -> snap_adc0/11(in_p1_d2)
  bus_expand1/4(out3) -> snap_adc0/12(in_p1_d3)
  bus_expand1/5(out2) -> snap_adc0/13(in_p1_d4_u8)
  bus_expand11/5(lsb_out1) -> snap_adc1/4(in_p1_d7)
  bus_expand11/4(out2) -> snap_adc1/3(in_p1_d6)
  bus_expand11/3(out3) -> snap_adc1/2(in_p1_d5)
  bus_expand11/2(out4) -> snap_adc1/1(in_p1_d4_l2)
  pipeline161/1(q) -> snap_adc0/14(we)
  gbe0/7(rx_valid) -> pipeline62/1(d)
  pipeline62/1(q) -> [forty_gbe_rx_valid]
  Counter1/1 -> pipeline165/1(d)
  pipeline165/1(q) -> sync80_count/1(out_reg)
  pipeline65/1(q) -> Counter1/1
  pipeline109/1(q) -> Counter1/2
  [sys_rst] -> edge_detect9/1(in)
  [sync80] -> edge_detect10/1(in)
  edge_detect9/1(out) -> pipeline65/1(d)
  edge_detect10/1(out) -> pipeline109/1(d)
  Convert/1 -> [f_per_x]
  [delay_sync] -> Mux4/2
  [sync80] -> Mux4/3
  [delay_d0] -> Mux3/2
  [d80_adc0] -> Mux3/3
  [delay_d1] -> Mux5/2
  [d80_adc1] -> Mux5/3
  [ct_d256] -> Delay16/1
  [ct_dv] -> Delay17/1
  [ct_sync] -> Delay18/1
  [valid80] -> Mux2/3
  [delay_dv] -> Mux2/2
  Delay33/1 -> pipeline139/1(d)
  Delay35/1 -> pipeline151/1(d)
  [hmc_data_p0] -> Concat5/1
  [hmc_data_p1] -> Concat5/2
  bus_expand2/1(msb_out2) -> [tg_data_p0]
  bus_expand2/2(lsb_out1) -> [tg_data_p1]
  control/14(in_gbe_stopmux) -> pipeline9/1(d)
  pipeline9/1(q) -> [gbe_stopmux]
  Constant33/1 -> concat1/2
  [flag_time] -> concat1/1
  [flag_sync] -> NEW_pack/1(sync_in)
  [flag_dvalid] -> NEW_pack/2(en)
  [flag_misc] -> NEW_pack/3(din)
  concat1/1 -> [pack_sync_time], NEW_pack/4(timestamp)
  [tx_board_id] -> NEW_pack/5(board_id)
  [tx_ip_base] -> NEW_pack/6(base_ip)
  [tx_port] -> NEW_pack/7(base_port)
  Constant32/1 -> NEW_pack/10(ips_per_destination)
  Constant30/1 -> NEW_pack/9(n_destinations)
  Constant28/1 -> NEW_pack/8(step_size)
  [flag_pktstart] -> NEW_pack/11(pkt_start)
  pipeline58/1(q) -> [s256_d]
  pipeline64/1(q) -> [s256_v]
  pipeline79/1(q) -> [s256_eof]
  pipeline94/1(q) -> [s256_of]
  pipeline95/1(q) -> [s256_ip]
  pipeline117/1(q) -> [s256_port]
  pipeline118/1(q) -> Terminator15/1
  NEW_pack/1(dout) -> pipeline58/1(d)
  NEW_pack/2(dvalid) -> pipeline64/1(d)
  NEW_pack/3(eof) -> pipeline79/1(d)
  NEW_pack/4(overflow) -> pipeline94/1(d)
  NEW_pack/5(destination_ip) -> pipeline95/1(d)
  NEW_pack/6(destination_port) -> pipeline117/1(d)
  NEW_pack/7(sync) -> pipeline118/1(d)
  Delay16/1 -> [ct_data]
  Delay17/1 -> [ct_dvalid]
  Delay18/1 -> [ct_s]
  x_setup/7(in_pktoffset_sel) -> pipeline63/1(d)
  pipeline63/1(q) -> [pktoffset_sel]
  control/15(in_pfb_bypass) -> pipeline66/1(d)
  pipeline66/1(q) -> [pfb_bypass]
  Delay21/1 -> cd_compensation0/1(sync_in)
  Delay22/1 -> cd_compensation0/3(en)
  Delay23/1 -> cd_compensation0/4(delay_val)
  Delay24/1 -> cd_compensation0/5(load_val)
  [dout_tl_cd0] -> Delay29/1
  Delay25/1 -> cd_compensation1/1(sync_in)
  Delay26/1 -> cd_compensation1/3(en)
  Delay27/1 -> cd_compensation1/4(delay_val)
  Delay28/1 -> cd_compensation1/5(load_val)
  pipeline134/1(q) -> [tl_cd0_arm]
  pipeline135/1(q) -> [tl_cd0_load_immediate]
  pipeline136/1(q) -> [tl_cd0_load_time]
  pipeline138/1(q) -> [tl_cd1_load_immediate]
  pipeline137/1(q) -> [tl_cd1_arm]
  pipeline143/1(q) -> [tl_cd1_load_time]
  [delay_d0] -> Slice13/1
  Delay29/1 -> cd_compensation0/2(din)
  Delay30/1 -> cd_compensation1/2(din)
  [dout_tl_cd0] -> Delay30/1
  ts_tvg/1(sync) -> pipeline10/1(d)
  ts_tvg/2(d160) -> pipeline11/1(d)
  ts_tvg/3(dv) -> pipeline12/1(d)
  ts_tvg/4(time) -> pipeline15/1(d)
  ts_tvg/5(recvd) -> pipeline17/1(d)
  control/16(in_ts_tvg_en) -> pipeline148/1(d)
  pipeline148/1(q) -> [ts_tvg_en]
  [ts_tvg_en] -> ts_tvg/1(tvg_en)
  [d80_adc0] -> Slice10/1
  pipeline145/1(q) -> snap_cd_time_debug/9(in_delay_data)
  pipeline133/1(q) -> snap_cd_time_debug/14(stop), snap_cd_time_debug/7(in_delay_sync)
  pipeline126/1(q) -> snap_cd_time_debug/3(in_unpack_data)
  pipeline123/1(q) -> snap_cd_time_debug/2(in_unpack_dv), snap_cd_time_debug/12(we)
  pipeline119/1(q) -> snap_cd_time_debug/1(in_unpack_sync)
  pipeline128/1(q) -> snap_cd_time_debug/5(in_d80valid)
  pipeline127/1(q) -> snap_cd_time_debug/4(in_d80sync), snap_cd_time_debug/13(trig)
  pipeline132/1(q) -> snap_cd_time_debug/6(in_data80)
  pipeline144/1(q) -> snap_cd_time_debug/8(in_delay_dv)
  [unpack_sync] -> pipeline119/1(d)
  [unpack_dv] -> pipeline123/1(d)
  [unpack_timestamp] -> pipeline126/1(d)
  Slice10/1 -> pipeline132/1(d)
  [valid80] -> pipeline128/1(d)
  [sync80] -> pipeline127/1(d)
  Slice13/1 -> pipeline145/1(d)
  [delay_dv] -> pipeline144/1(d)
  [delay_sync] -> pipeline133/1(d)
  [cd_error_p1] -> Subsystem2/3(in1)
  Subsystem2/2(out1) -> cd_status/2(out_pol1_err_cnt)
